simulink model "REFvsFI"  (R2023a)
settings: Solver=FixedStepAuto  StartTime=0.0  StopTime=T  RelTol=1e-3  EnableMultiTasking=on
values from neighbouring files (symbols this model uses):
  Ts = 1    [TestDataGen.m]
libraries: My_FI_Operations x114, simulink x2
(part 2 of 5)

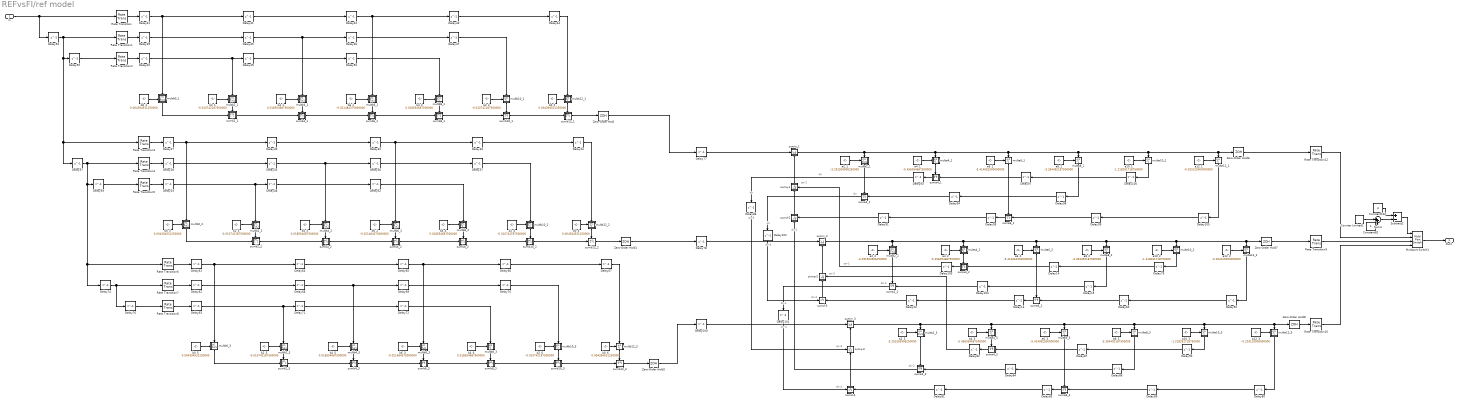
== system REFvsFI/ref model ==
  note: dn-1
  note: dn-2
  note: qn-3
  note: dn-3
  note: qn
  note: dn
  note: dn-4
  note: dn-2
  note: dn-1
  note: qn
  note: dn-4
  note: dn
  note: dn-3
  note: qn-2
  note: qn-3
  note: qn-1
  note: qn-1
  in : Inport
  Constant102 : Constant  Value=4
  Constant82 : Constant
  Counter Limited1 : simulink/Sources/Counter Limited  uplimit=2  tsamp=Ts
  Delay{13..15,23,27..37,39..50,52,60..72,75,77..78,80..82,84..95,97..105,109} (69 alike) : Delay  DelayLength=1  SampleTime=3*Ts
  Delay{53,55,57,59,74,76} (6 alike) : Delay  DelayLength=1  SampleTime=Ts
  Multiport Switch1 : MultiPortSwitch  OutDataTypeStr=double  RndMeth=Nearest  SaturateOnIntegerOverflow=off  InputSameDT=off
  Rate Transition{,1..8} (9 alike) : RateTransition  OutPortSampleTime=3*Ts
  Rate Transition10 : RateTransition  OutPortSampleTime=Ts
  Rate Transition12 : RateTransition  OutPortSampleTime=Ts
  Rate Transition9 : RateTransition  OutPortSampleTime=Ts
  Subtract2 : Sum  Inputs=+-
  Sum4 : Sum  Inputs=|++
  Zero-Order Hold{,1..2,6..8} (6 alike) : ZeroOrderHold  SampleTime=3*Ts
  a10_1 : Constant  Value=-1.218261718750000  OutDataTypeStr=double
  a10_2 : Constant  Value=-1.218261718750000  OutDataTypeStr=double
  a10_3 : Constant  Value=-1.218261718750000  OutDataTypeStr=double
  a12_1 : Constant  Value=-0.203125000000000  OutDataTypeStr=double
  a12_2 : Constant  Value=-0.203125000000000  OutDataTypeStr=double
  a12_3 : Constant  Value=-0.203125000000000  OutDataTypeStr=double
  a2_1 : Constant  Value=-3.291503906250000  OutDataTypeStr=double
  a2_2 : Constant  Value=-3.291503906250000  OutDataTypeStr=double
  a2_3 : Constant  Value=-3.291503906250000  OutDataTypeStr=double
  a4_1 : Constant  Value=-5.456054687500000  OutDataTypeStr=double
  a4_2 : Constant  Value=-5.456054687500000  OutDataTypeStr=double
  a4_3 : Constant  Value=-5.456054687500000  OutDataTypeStr=double
  a6_1 : Constant  Value=-5.414062500000000  OutDataTypeStr=double
  a6_2 : Constant  Value=-5.414062500000000  OutDataTypeStr=double
  a6_3 : Constant  Value=-5.414062500000000  OutDataTypeStr=double
  a8_1 : Constant  Value=-3.354492187500000  OutDataTypeStr=double
  a8_2 : Constant  Value=-3.354492187500000  OutDataTypeStr=double
  a8_3 : Constant  Value=-3.354492187500000  OutDataTypeStr=double
  b0_{1..6} (6 alike) : Constant  Value=0.004394531250000  OutDataTypeStr=double
  b2_{1..6} (6 alike) : Constant  Value=-0.010742187500000  OutDataTypeStr=double
  b4_{1..6} (6 alike) : Constant  Value=0.018554687500000  OutDataTypeStr=double
  b6_1 : Constant  Value=-0.021484375000000  OutDataTypeStr=double
  b6_2 : Constant  Value=-0.021484375000000  OutDataTypeStr=double
  b6_3 : Constant  Value=-0.021484375000000  OutDataTypeStr=double
  multa10_1 : Subsystem  AncestorBlock=My_FI_Operations/multa10_
      settings: LibrarySourceBlock=My_FI_Operations/multa10_  PortSchema="{\"entries\":[{\"content\":{\"sides\":[{\"content\":{\"connectorIds\":[\"In1\"]},\"type\":\"ConnectorPlacement.EquallySpacedRectSide\",\"uuid\":\"423828e0-6700-4575-ac06-a5fb7cb5569f\"},{\"content\":{\"connectorIds\":[],\"side\":\"RIGHT\"},\"type\":\"ConnectorPlacement.EquallySpacedRectSide\",\"uuid\":\"a42db842-eb55-44f2-8f04-0144bc45d908\"},{\"content\":{\"connectorIds\":[\"In2\"],\"side\":\"TOP\"},\"type\":\"ConnectorPlacement.EquallySpacedRectSide\",\"uuid\":\"eef5137d-31f0-46b4-a53b-5aa31464a7f9\"},{\"content\":{\"connectorIds\":[\"Out1\"],\"side\":\"BOTTOM\"},\"type\":\"ConnectorPlacement.EquallySpacedRectSide\",\"uuid\":\"0c804fa9-8d94-49f3-91d8-5fb511150c33\"}]},\"type\":\"ConnectorPlacement.EquallySpacedConnector\",\"uuid\":\"7dd7fe03-b221-4701-a7b2-6552f08320da\"}],\"packageUris\":[\"http://schema.mathworks.com/mf0/Connector/R2020b\"],\"version\":\"1.0\"}"
      mask Display: disp('x')
  multa10_2 : Subsystem  AncestorBlock=My_FI_Operations/multa10_
      settings: LibrarySourceBlock=My_FI_Operations/multa10_  PortSchema="{\"entries\":[{\"content\":{\"sides\":[{\"content\":{\"connectorIds\":[\"In1\"]},\"type\":\"ConnectorPlacement.EquallySpacedRectSide\",\"uuid\":\"423828e0-6700-4575-ac06-a5fb7cb5569f\"},{\"content\":{\"connectorIds\":[],\"side\":\"RIGHT\"},\"type\":\"ConnectorPlacement.EquallySpacedRectSide\",\"uuid\":\"a42db842-eb55-44f2-8f04-0144bc45d908\"},{\"content\":{\"connectorIds\":[\"In2\"],\"side\":\"TOP\"},\"type\":\"ConnectorPlacement.EquallySpacedRectSide\",\"uuid\":\"eef5137d-31f0-46b4-a53b-5aa31464a7f9\"},{\"content\":{\"connectorIds\":[\"Out1\"],\"side\":\"BOTTOM\"},\"type\":\"ConnectorPlacement.EquallySpacedRectSide\",\"uuid\":\"0c804fa9-8d94-49f3-91d8-5fb511150c33\"}]},\"type\":\"ConnectorPlacement.EquallySpacedConnector\",\"uuid\":\"7dd7fe03-b221-4701-a7b2-6552f08320da\"}],\"packageUris\":[\"http://schema.mathworks.com/mf0/Connector/R2020b\"],\"version\":\"1.0\"}"
      mask Display: disp('x')
  multa10_3 : Subsystem  AncestorBlock=My_FI_Operations/multa10_
      settings: LibrarySourceBlock=My_FI_Operations/multa10_  PortSchema="{\"entries\":[{\"content\":{\"sides\":[{\"content\":{\"connectorIds\":[\"In1\"]},\"type\":\"ConnectorPlacement.EquallySpacedRectSide\",\"uuid\":\"423828e0-6700-4575-ac06-a5fb7cb5569f\"},{\"content\":{\"connectorIds\":[],\"side\":\"RIGHT\"},\"type\":\"ConnectorPlacement.EquallySpacedRectSide\",\"uuid\":\"a42db842-eb55-44f2-8f04-0144bc45d908\"},{\"content\":{\"connectorIds\":[\"In2\"],\"side\":\"TOP\"},\"type\":\"ConnectorPlacement.EquallySpacedRectSide\",\"uuid\":\"eef5137d-31f0-46b4-a53b-5aa31464a7f9\"},{\"content\":{\"connectorIds\":[\"Out1\"],\"side\":\"BOTTOM\"},\"type\":\"ConnectorPlacement.EquallySpacedRectSide\",\"uuid\":\"0c804fa9-8d94-49f3-91d8-5fb511150c33\"}]},\"type\":\"ConnectorPlacement.EquallySpacedConnector\",\"uuid\":\"7dd7fe03-b221-4701-a7b2-6552f08320da\"}],\"packageUris\":[\"http://schema.mathworks.com/mf0/Connector/R2020b\"],\"version\":\"1.0\"}"
      mask Display: disp('x')
  multa12_1 : Subsystem  AncestorBlock=My_FI_Operations/multa12_
      settings: LibrarySourceBlock=My_FI_Operations/multa12_  PortSchema="{\"entries\":[{\"content\":{\"sides\":[{\"content\":{\"connectorIds\":[\"In1\"]},\"type\":\"ConnectorPlacement.EquallySpacedRectSide\",\"uuid\":\"423828e0-6700-4575-ac06-a5fb7cb5569f\"},{\"content\":{\"connectorIds\":[],\"side\":\"RIGHT\"},\"type\":\"ConnectorPlacement.EquallySpacedRectSide\",\"uuid\":\"a42db842-eb55-44f2-8f04-0144bc45d908\"},{\"content\":{\"connectorIds\":[\"In2\"],\"side\":\"TOP\"},\"type\":\"ConnectorPlacement.EquallySpacedRectSide\",\"uuid\":\"eef5137d-31f0-46b4-a53b-5aa31464a7f9\"},{\"content\":{\"connectorIds\":[\"Out1\"],\"side\":\"BOTTOM\"},\"type\":\"ConnectorPlacement.EquallySpacedRectSide\",\"uuid\":\"8449918d-02c6-4967-8b4f-9e277713318d\"}]},\"type\":\"ConnectorPlacement.EquallySpacedConnector\",\"uuid\":\"7dd7fe03-b221-4701-a7b2-6552f08320da\"}],\"packageUris\":[\"http://schema.mathworks.com/mf0/Connector/R2020b\"],\"version\":\"1.0\"}"
      mask Display: disp('x')
  multa12_2 : Subsystem  AncestorBlock=My_FI_Operations/multa12_
      settings: LibrarySourceBlock=My_FI_Operations/multa12_  PortSchema="{\"entries\":[{\"content\":{\"sides\":[{\"content\":{\"connectorIds\":[\"In1\"]},\"type\":\"ConnectorPlacement.EquallySpacedRectSide\",\"uuid\":\"423828e0-6700-4575-ac06-a5fb7cb5569f\"},{\"content\":{\"connectorIds\":[],\"side\":\"RIGHT\"},\"type\":\"ConnectorPlacement.EquallySpacedRectSide\",\"uuid\":\"a42db842-eb55-44f2-8f04-0144bc45d908\"},{\"content\":{\"connectorIds\":[\"In2\"],\"side\":\"TOP\"},\"type\":\"ConnectorPlacement.EquallySpacedRectSide\",\"uuid\":\"eef5137d-31f0-46b4-a53b-5aa31464a7f9\"},{\"content\":{\"connectorIds\":[\"Out1\"],\"side\":\"BOTTOM\"},\"type\":\"ConnectorPlacement.EquallySpacedRectSide\",\"uuid\":\"8449918d-02c6-4967-8b4f-9e277713318d\"}]},\"type\":\"ConnectorPlacement.EquallySpacedConnector\",\"uuid\":\"7dd7fe03-b221-4701-a7b2-6552f08320da\"}],\"packageUris\":[\"http://schema.mathworks.com/mf0/Connector/R2020b\"],\"version\":\"1.0\"}"
      mask Display: disp('x')
  multa12_3 : Subsystem  AncestorBlock=My_FI_Operations/multa12_
      settings: LibrarySourceBlock=My_FI_Operations/multa12_  PortSchema="{\"entries\":[{\"content\":{\"sides\":[{\"content\":{\"connectorIds\":[\"In1\"]},\"type\":\"ConnectorPlacement.EquallySpacedRectSide\",\"uuid\":\"423828e0-6700-4575-ac06-a5fb7cb5569f\"},{\"content\":{\"connectorIds\":[],\"side\":\"RIGHT\"},\"type\":\"ConnectorPlacement.EquallySpacedRectSide\",\"uuid\":\"a42db842-eb55-44f2-8f04-0144bc45d908\"},{\"content\":{\"connectorIds\":[\"In2\"],\"side\":\"TOP\"},\"type\":\"ConnectorPlacement.EquallySpacedRectSide\",\"uuid\":\"eef5137d-31f0-46b4-a53b-5aa31464a7f9\"},{\"content\":{\"connectorIds\":[\"Out1\"],\"side\":\"BOTTOM\"},\"type\":\"ConnectorPlacement.EquallySpacedRectSide\",\"uuid\":\"8449918d-02c6-4967-8b4f-9e277713318d\"}]},\"type\":\"ConnectorPlacement.EquallySpacedConnector\",\"uuid\":\"7dd7fe03-b221-4701-a7b2-6552f08320da\"}],\"packageUris\":[\"http://schema.mathworks.com/mf0/Connector/R2020b\"],\"version\":\"1.0\"}"
      mask Display: disp('x')
  multa2_1 : Subsystem  AncestorBlock=My_FI_Operations/multa2_
      settings: LibrarySourceBlock=My_FI_Operations/multa2_  PortSchema="{\"entries\":[{\"content\":{\"sides\":[{\"content\":{\"connectorIds\":[\"In1\"]},\"type\":\"ConnectorPlacement.EquallySpacedRectSide\",\"uuid\":\"423828e0-6700-4575-ac06-a5fb7cb5569f\"},{\"content\":{\"connectorIds\":[],\"side\":\"RIGHT\"},\"type\":\"ConnectorPlacement.EquallySpacedRectSide\",\"uuid\":\"a42db842-eb55-44f2-8f04-0144bc45d908\"},{\"content\":{\"connectorIds\":[\"In2\"],\"side\":\"TOP\"},\"type\":\"ConnectorPlacement.EquallySpacedRectSide\",\"uuid\":\"eef5137d-31f0-46b4-a53b-5aa31464a7f9\"},{\"content\":{\"connectorIds\":[\"Out1\"],\"side\":\"BOTTOM\"},\"type\":\"ConnectorPlacement.EquallySpacedRectSide\",\"uuid\":\"55d96b2a-2b7e-4fdf-a401-8e78f7d2a1aa\"}]},\"type\":\"ConnectorPlacement.EquallySpacedConnector\",\"uuid\":\"7dd7fe03-b221-4701-a7b2-6552f08320da\"}],\"packageUris\":[\"http://schema.mathworks.com/mf0/Connector/R2020b\"],\"version\":\"1.0\"}"
      mask Display: disp('x')
  multa2_2 : Subsystem  AncestorBlock=My_FI_Operations/multa2_
      settings: LibrarySourceBlock=My_FI_Operations/multa2_  PortSchema="{\"entries\":[{\"content\":{\"sides\":[{\"content\":{\"connectorIds\":[\"In1\"]},\"type\":\"ConnectorPlacement.EquallySpacedRectSide\",\"uuid\":\"423828e0-6700-4575-ac06-a5fb7cb5569f\"},{\"content\":{\"connectorIds\":[],\"side\":\"RIGHT\"},\"type\":\"ConnectorPlacement.EquallySpacedRectSide\",\"uuid\":\"a42db842-eb55-44f2-8f04-0144bc45d908\"},{\"content\":{\"connectorIds\":[\"In2\"],\"side\":\"TOP\"},\"type\":\"ConnectorPlacement.EquallySpacedRectSide\",\"uuid\":\"eef5137d-31f0-46b4-a53b-5aa31464a7f9\"},{\"content\":{\"connectorIds\":[\"Out1\"],\"side\":\"BOTTOM\"},\"type\":\"ConnectorPlacement.EquallySpacedRectSide\",\"uuid\":\"55d96b2a-2b7e-4fdf-a401-8e78f7d2a1aa\"}]},\"type\":\"ConnectorPlacement.EquallySpacedConnector\",\"uuid\":\"7dd7fe03-b221-4701-a7b2-6552f08320da\"}],\"packageUris\":[\"http://schema.mathworks.com/mf0/Connector/R2020b\"],\"version\":\"1.0\"}"
      mask Display: disp('x')
  multa2_3 : Subsystem  AncestorBlock=My_FI_Operations/multa2_
      settings: LibrarySourceBlock=My_FI_Operations/multa2_  PortSchema="{\"entries\":[{\"content\":{\"sides\":[{\"content\":{\"connectorIds\":[\"In1\"]},\"type\":\"ConnectorPlacement.EquallySpacedRectSide\",\"uuid\":\"423828e0-6700-4575-ac06-a5fb7cb5569f\"},{\"content\":{\"connectorIds\":[],\"side\":\"RIGHT\"},\"type\":\"ConnectorPlacement.EquallySpacedRectSide\",\"uuid\":\"a42db842-eb55-44f2-8f04-0144bc45d908\"},{\"content\":{\"connectorIds\":[\"In2\"],\"side\":\"TOP\"},\"type\":\"ConnectorPlacement.EquallySpacedRectSide\",\"uuid\":\"eef5137d-31f0-46b4-a53b-5aa31464a7f9\"},{\"content\":{\"connectorIds\":[\"Out1\"],\"side\":\"BOTTOM\"},\"type\":\"ConnectorPlacement.EquallySpacedRectSide\",\"uuid\":\"55d96b2a-2b7e-4fdf-a401-8e78f7d2a1aa\"}]},\"type\":\"ConnectorPlacement.EquallySpacedConnector\",\"uuid\":\"7dd7fe03-b221-4701-a7b2-6552f08320da\"}],\"packageUris\":[\"http://schema.mathworks.com/mf0/Connector/R2020b\"],\"version\":\"1.0\"}"
      mask Display: disp('x')
  multa4_1 : Subsystem  AncestorBlock=My_FI_Operations/multa4_
      settings: LibrarySourceBlock=My_FI_Operations/multa4_  PortSchema="{\"entries\":[{\"content\":{\"sides\":[{\"content\":{\"connectorIds\":[\"In1\"]},\"type\":\"ConnectorPlacement.EquallySpacedRectSide\",\"uuid\":\"423828e0-6700-4575-ac06-a5fb7cb5569f\"},{\"content\":{\"connectorIds\":[],\"side\":\"RIGHT\"},\"type\":\"ConnectorPlacement.EquallySpacedRectSide\",\"uuid\":\"a42db842-eb55-44f2-8f04-0144bc45d908\"},{\"content\":{\"connectorIds\":[\"In2\"],\"side\":\"TOP\"},\"type\":\"ConnectorPlacement.EquallySpacedRectSide\",\"uuid\":\"eef5137d-31f0-46b4-a53b-5aa31464a7f9\"},{\"content\":{\"connectorIds\":[\"Out1\"],\"side\":\"BOTTOM\"},\"type\":\"ConnectorPlacement.EquallySpacedRectSide\",\"uuid\":\"24a9476e-4370-431a-bbc5-245c90c7a6e7\"}]},\"type\":\"ConnectorPlacement.EquallySpacedConnector\",\"uuid\":\"7dd7fe03-b221-4701-a7b2-6552f08320da\"}],\"packageUris\":[\"http://schema.mathworks.com/mf0/Connector/R2020b\"],\"version\":\"1.0\"}"
      mask Display: disp('x')
  multa4_2 : Subsystem  AncestorBlock=My_FI_Operations/multa4_
      settings: LibrarySourceBlock=My_FI_Operations/multa4_  PortSchema="{\"entries\":[{\"content\":{\"sides\":[{\"content\":{\"connectorIds\":[\"In1\"]},\"type\":\"ConnectorPlacement.EquallySpacedRectSide\",\"uuid\":\"423828e0-6700-4575-ac06-a5fb7cb5569f\"},{\"content\":{\"connectorIds\":[],\"side\":\"RIGHT\"},\"type\":\"ConnectorPlacement.EquallySpacedRectSide\",\"uuid\":\"a42db842-eb55-44f2-8f04-0144bc45d908\"},{\"content\":{\"connectorIds\":[\"In2\"],\"side\":\"TOP\"},\"type\":\"ConnectorPlacement.EquallySpacedRectSide\",\"uuid\":\"eef5137d-31f0-46b4-a53b-5aa31464a7f9\"},{\"content\":{\"connectorIds\":[\"Out1\"],\"side\":\"BOTTOM\"},\"type\":\"ConnectorPlacement.EquallySpacedRectSide\",\"uuid\":\"24a9476e-4370-431a-bbc5-245c90c7a6e7\"}]},\"type\":\"ConnectorPlacement.EquallySpacedConnector\",\"uuid\":\"7dd7fe03-b221-4701-a7b2-6552f08320da\"}],\"packageUris\":[\"http://schema.mathworks.com/mf0/Connector/R2020b\"],\"version\":\"1.0\"}"
      mask Display: disp('x')
  multa4_3 : Subsystem  AncestorBlock=My_FI_Operations/multa4_
      settings: LibrarySourceBlock=My_FI_Operations/multa4_  PortSchema="{\"entries\":[{\"content\":{\"sides\":[{\"content\":{\"connectorIds\":[\"In1\"]},\"type\":\"ConnectorPlacement.EquallySpacedRectSide\",\"uuid\":\"423828e0-6700-4575-ac06-a5fb7cb5569f\"},{\"content\":{\"connectorIds\":[],\"side\":\"RIGHT\"},\"type\":\"ConnectorPlacement.EquallySpacedRectSide\",\"uuid\":\"a42db842-eb55-44f2-8f04-0144bc45d908\"},{\"content\":{\"connectorIds\":[\"In2\"],\"side\":\"TOP\"},\"type\":\"ConnectorPlacement.EquallySpacedRectSide\",\"uuid\":\"eef5137d-31f0-46b4-a53b-5aa31464a7f9\"},{\"content\":{\"connectorIds\":[\"Out1\"],\"side\":\"BOTTOM\"},\"type\":\"ConnectorPlacement.EquallySpacedRectSide\",\"uuid\":\"24a9476e-4370-431a-bbc5-245c90c7a6e7\"}]},\"type\":\"ConnectorPlacement.EquallySpacedConnector\",\"uuid\":\"7dd7fe03-b221-4701-a7b2-6552f08320da\"}],\"packageUris\":[\"http://schema.mathworks.com/mf0/Connector/R2020b\"],\"version\":\"1.0\"}"
      mask Display: disp('x')
  multa6_1 : Subsystem  AncestorBlock=My_FI_Operations/multa6_
      settings: LibrarySourceBlock=My_FI_Operations/multa6_  PortSchema="{\"entries\":[{\"content\":{\"sides\":[{\"content\":{\"connectorIds\":[\"In1\"]},\"type\":\"ConnectorPlacement.EquallySpacedRectSide\",\"uuid\":\"423828e0-6700-4575-ac06-a5fb7cb5569f\"},{\"content\":{\"connectorIds\":[],\"side\":\"RIGHT\"},\"type\":\"ConnectorPlacement.EquallySpacedRectSide\",\"uuid\":\"a42db842-eb55-44f2-8f04-0144bc45d908\"},{\"content\":{\"connectorIds\":[\"In2\"],\"side\":\"TOP\"},\"type\":\"ConnectorPlacement.EquallySpacedRectSide\",\"uuid\":\"eef5137d-31f0-46b4-a53b-5aa31464a7f9\"},{\"content\":{\"connectorIds\":[\"Out1\"],\"side\":\"BOTTOM\"},\"type\":\"ConnectorPlacement.EquallySpacedRectSide\",\"uuid\":\"47329aef-84bb-47a0-9b32-b12909a392a1\"}]},\"type\":\"ConnectorPlacement.EquallySpacedConnector\",\"uuid\":\"7dd7fe03-b221-4701-a7b2-6552f08320da\"}],\"packageUris\":[\"http://schema.mathworks.com/mf0/Connector/R2020b\"],\"version\":\"1.0\"}"
      mask Display: disp('x')
  multa6_2 : Subsystem  AncestorBlock=My_FI_Operations/multa6_
      settings: LibrarySourceBlock=My_FI_Operations/multa6_  PortSchema="{\"entries\":[{\"content\":{\"sides\":[{\"content\":{\"connectorIds\":[\"In1\"]},\"type\":\"ConnectorPlacement.EquallySpacedRectSide\",\"uuid\":\"423828e0-6700-4575-ac06-a5fb7cb5569f\"},{\"content\":{\"connectorIds\":[],\"side\":\"RIGHT\"},\"type\":\"ConnectorPlacement.EquallySpacedRectSide\",\"uuid\":\"a42db842-eb55-44f2-8f04-0144bc45d908\"},{\"content\":{\"connectorIds\":[\"In2\"],\"side\":\"TOP\"},\"type\":\"ConnectorPlacement.EquallySpacedRectSide\",\"uuid\":\"eef5137d-31f0-46b4-a53b-5aa31464a7f9\"},{\"content\":{\"connectorIds\":[\"Out1\"],\"side\":\"BOTTOM\"},\"type\":\"ConnectorPlacement.EquallySpacedRectSide\",\"uuid\":\"47329aef-84bb-47a0-9b32-b12909a392a1\"}]},\"type\":\"ConnectorPlacement.EquallySpacedConnector\",\"uuid\":\"7dd7fe03-b221-4701-a7b2-6552f08320da\"}],\"packageUris\":[\"http://schema.mathworks.com/mf0/Connector/R2020b\"],\"version\":\"1.0\"}"
      mask Display: disp('x')
  multa6_3 : Subsystem  AncestorBlock=My_FI_Operations/multa6_
      settings: LibrarySourceBlock=My_FI_Operations/multa6_  PortSchema="{\"entries\":[{\"content\":{\"sides\":[{\"content\":{\"connectorIds\":[\"In1\"]},\"type\":\"ConnectorPlacement.EquallySpacedRectSide\",\"uuid\":\"423828e0-6700-4575-ac06-a5fb7cb5569f\"},{\"content\":{\"connectorIds\":[],\"side\":\"RIGHT\"},\"type\":\"ConnectorPlacement.EquallySpacedRectSide\",\"uuid\":\"a42db842-eb55-44f2-8f04-0144bc45d908\"},{\"content\":{\"connectorIds\":[\"In2\"],\"side\":\"TOP\"},\"type\":\"ConnectorPlacement.EquallySpacedRectSide\",\"uuid\":\"eef5137d-31f0-46b4-a53b-5aa31464a7f9\"},{\"content\":{\"connectorIds\":[\"Out1\"],\"side\":\"BOTTOM\"},\"type\":\"ConnectorPlacement.EquallySpacedRectSide\",\"uuid\":\"47329aef-84bb-47a0-9b32-b12909a392a1\"}]},\"type\":\"ConnectorPlacement.EquallySpacedConnector\",\"uuid\":\"7dd7fe03-b221-4701-a7b2-6552f08320da\"}],\"packageUris\":[\"http://schema.mathworks.com/mf0/Connector/R2020b\"],\"version\":\"1.0\"}"
      mask Display: disp('x')
  multa8_1 : Subsystem  AncestorBlock=My_FI_Operations/multa8_
      settings: LibrarySourceBlock=My_FI_Operations/multa8_  PortSchema="{\"entries\":[{\"content\":{\"sides\":[{\"content\":{\"connectorIds\":[\"In1\"]},\"type\":\"ConnectorPlacement.EquallySpacedRectSide\",\"uuid\":\"423828e0-6700-4575-ac06-a5fb7cb5569f\"},{\"content\":{\"connectorIds\":[],\"side\":\"RIGHT\"},\"type\":\"ConnectorPlacement.EquallySpacedRectSide\",\"uuid\":\"a42db842-eb55-44f2-8f04-0144bc45d908\"},{\"content\":{\"connectorIds\":[\"In2\"],\"side\":\"TOP\"},\"type\":\"ConnectorPlacement.EquallySpacedRectSide\",\"uuid\":\"eef5137d-31f0-46b4-a53b-5aa31464a7f9\"},{\"content\":{\"connectorIds\":[\"Out1\"],\"side\":\"BOTTOM\"},\"type\":\"ConnectorPlacement.EquallySpacedRectSide\",\"uuid\":\"5c073f60-f22f-4cd7-abc5-d0d5f88f0213\"}]},\"type\":\"ConnectorPlacement.EquallySpacedConnector\",\"uuid\":\"7dd7fe03-b221-4701-a7b2-6552f08320da\"}],\"packageUris\":[\"http://schema.mathworks.com/mf0/Connector/R2020b\"],\"version\":\"1.0\"}"
      mask Display: disp('x')
  multa8_2 : Subsystem  AncestorBlock=My_FI_Operations/multa8_
      settings: LibrarySourceBlock=My_FI_Operations/multa8_  PortSchema="{\"entries\":[{\"content\":{\"sides\":[{\"content\":{\"connectorIds\":[\"In1\"]},\"type\":\"ConnectorPlacement.EquallySpacedRectSide\",\"uuid\":\"423828e0-6700-4575-ac06-a5fb7cb5569f\"},{\"content\":{\"connectorIds\":[],\"side\":\"RIGHT\"},\"type\":\"ConnectorPlacement.EquallySpacedRectSide\",\"uuid\":\"a42db842-eb55-44f2-8f04-0144bc45d908\"},{\"content\":{\"connectorIds\":[\"In2\"],\"side\":\"TOP\"},\"type\":\"ConnectorPlacement.EquallySpacedRectSide\",\"uuid\":\"eef5137d-31f0-46b4-a53b-5aa31464a7f9\"},{\"content\":{\"connectorIds\":[\"Out1\"],\"side\":\"BOTTOM\"},\"type\":\"ConnectorPlacement.EquallySpacedRectSide\",\"uuid\":\"5c073f60-f22f-4cd7-abc5-d0d5f88f0213\"}]},\"type\":\"ConnectorPlacement.EquallySpacedConnector\",\"uuid\":\"7dd7fe03-b221-4701-a7b2-6552f08320da\"}],\"packageUris\":[\"http://schema.mathworks.com/mf0/Connector/R2020b\"],\"version\":\"1.0\"}"
      mask Display: disp('x')
  multa8_3 : Subsystem  AncestorBlock=My_FI_Operations/multa8_
      settings: LibrarySourceBlock=My_FI_Operations/multa8_  PortSchema="{\"entries\":[{\"content\":{\"sides\":[{\"content\":{\"connectorIds\":[\"In1\"]},\"type\":\"ConnectorPlacement.EquallySpacedRectSide\",\"uuid\":\"423828e0-6700-4575-ac06-a5fb7cb5569f\"},{\"content\":{\"connectorIds\":[],\"side\":\"RIGHT\"},\"type\":\"ConnectorPlacement.EquallySpacedRectSide\",\"uuid\":\"a42db842-eb55-44f2-8f04-0144bc45d908\"},{\"content\":{\"connectorIds\":[\"In2\"],\"side\":\"TOP\"},\"type\":\"ConnectorPlacement.EquallySpacedRectSide\",\"uuid\":\"eef5137d-31f0-46b4-a53b-5aa31464a7f9\"},{\"content\":{\"connectorIds\":[\"Out1\"],\"side\":\"BOTTOM\"},\"type\":\"ConnectorPlacement.EquallySpacedRectSide\",\"uuid\":\"5c073f60-f22f-4cd7-abc5-d0d5f88f0213\"}]},\"type\":\"ConnectorPlacement.EquallySpacedConnector\",\"uuid\":\"7dd7fe03-b221-4701-a7b2-6552f08320da\"}],\"packageUris\":[\"http://schema.mathworks.com/mf0/Connector/R2020b\"],\"version\":\"1.0\"}"
      mask Display: disp('x')
  multb0_1 : Subsystem  AncestorBlock=My_FI_Operations/multb0_
      settings: LibrarySourceBlock=My_FI_Operations/multb0_  PortSchema="{\"entries\":[{\"content\":{\"sides\":[{\"content\":{\"connectorIds\":[\"In1\"]},\"type\":\"ConnectorPlacement.EquallySpacedRectSide\",\"uuid\":\"20461ecc-945a-453b-bec8-f18bcbd4d7ca\"},{\"content\":{\"connectorIds\":[],\"side\":\"RIGHT\"},\"type\":\"ConnectorPlacement.EquallySpacedRectSide\",\"uuid\":\"a806ae65-26a1-4387-823f-a90265b6c751\"},{\"content\":{\"connectorIds\":[\"In2\"],\"side\":\"TOP\"},\"type\":\"ConnectorPlacement.EquallySpacedRectSide\",\"uuid\":\"faa34e1a-fdc6-4b39-b604-acf00955d353\"},{\"content\":{\"connectorIds\":[\"Out1\"],\"side\":\"BOTTOM\"},\"type\":\"ConnectorPlacement.EquallySpacedRectSide\",\"uuid\":\"6d48c7d1-ec45-4610-bf5d-3af7cf103011\"}]},\"type\":\"ConnectorPlacement.EquallySpacedConnector\",\"uuid\":\"f3c21808-e34e-4785-8275-0070ba5b450f\"}],\"packageUris\":[\"http://schema.mathworks.com/mf0/Connector/R2020b\"],\"version\":\"1.0\"}"
      mask Display: disp('x')
  multb0_2 : Subsystem  AncestorBlock=My_FI_Operations/multb0_
      settings: LibrarySourceBlock=My_FI_Operations/multb0_  PortSchema="{\"entries\":[{\"content\":{\"sides\":[{\"content\":{\"connectorIds\":[\"In1\"]},\"type\":\"ConnectorPlacement.EquallySpacedRectSide\",\"uuid\":\"20461ecc-945a-453b-bec8-f18bcbd4d7ca\"},{\"content\":{\"connectorIds\":[],\"side\":\"RIGHT\"},\"type\":\"ConnectorPlacement.EquallySpacedRectSide\",\"uuid\":\"a806ae65-26a1-4387-823f-a90265b6c751\"},{\"content\":{\"connectorIds\":[\"In2\"],\"side\":\"TOP\"},\"type\":\"ConnectorPlacement.EquallySpacedRectSide\",\"uuid\":\"faa34e1a-fdc6-4b39-b604-acf00955d353\"},{\"content\":{\"connectorIds\":[\"Out1\"],\"side\":\"BOTTOM\"},\"type\":\"ConnectorPlacement.EquallySpacedRectSide\",\"uuid\":\"6d48c7d1-ec45-4610-bf5d-3af7cf103011\"}]},\"type\":\"ConnectorPlacement.EquallySpacedConnector\",\"uuid\":\"f3c21808-e34e-4785-8275-0070ba5b450f\"}],\"packageUris\":[\"http://schema.mathworks.com/mf0/Connector/R2020b\"],\"version\":\"1.0\"}"
      mask Display: disp('x')
  multb0_3 : Subsystem  AncestorBlock=My_FI_Operations/multb0_
      settings: LibrarySourceBlock=My_FI_Operations/multb0_  PortSchema="{\"entries\":[{\"content\":{\"sides\":[{\"content\":{\"connectorIds\":[\"In1\"]},\"type\":\"ConnectorPlacement.EquallySpacedRectSide\",\"uuid\":\"20461ecc-945a-453b-bec8-f18bcbd4d7ca\"},{\"content\":{\"connectorIds\":[],\"side\":\"RIGHT\"},\"type\":\"ConnectorPlacement.EquallySpacedRectSide\",\"uuid\":\"a806ae65-26a1-4387-823f-a90265b6c751\"},{\"content\":{\"connectorIds\":[\"In2\"],\"side\":\"TOP\"},\"type\":\"ConnectorPlacement.EquallySpacedRectSide\",\"uuid\":\"faa34e1a-fdc6-4b39-b604-acf00955d353\"},{\"content\":{\"connectorIds\":[\"Out1\"],\"side\":\"BOTTOM\"},\"type\":\"ConnectorPlacement.EquallySpacedRectSide\",\"uuid\":\"6d48c7d1-ec45-4610-bf5d-3af7cf103011\"}]},\"type\":\"ConnectorPlacement.EquallySpacedConnector\",\"uuid\":\"f3c21808-e34e-4785-8275-0070ba5b450f\"}],\"packageUris\":[\"http://schema.mathworks.com/mf0/Connector/R2020b\"],\"version\":\"1.0\"}"
      mask Display: disp('x')
  multb10_1 : Subsystem  AncestorBlock=My_FI_Operations/multb10_
      settings: LibrarySourceBlock=My_FI_Operations/multb10_  PortSchema="{\"entries\":[{\"content\":{\"sides\":[{\"content\":{\"connectorIds\":[\"In1\"]},\"type\":\"ConnectorPlacement.EquallySpacedRectSide\",\"uuid\":\"20461ecc-945a-453b-bec8-f18bcbd4d7ca\"},{\"content\":{\"connectorIds\":[],\"side\":\"RIGHT\"},\"type\":\"ConnectorPlacement.EquallySpacedRectSide\",\"uuid\":\"a806ae65-26a1-4387-823f-a90265b6c751\"},{\"content\":{\"connectorIds\":[\"In2\"],\"side\":\"TOP\"},\"type\":\"ConnectorPlacement.EquallySpacedRectSide\",\"uuid\":\"faa34e1a-fdc6-4b39-b604-acf00955d353\"},{\"content\":{\"connectorIds\":[\"Out1\"],\"side\":\"BOTTOM\"},\"type\":\"ConnectorPlacement.EquallySpacedRectSide\",\"uuid\":\"227775b0-b587-499e-95de-63528f3ed159\"}]},\"type\":\"ConnectorPlacement.EquallySpacedConnector\",\"uuid\":\"f3c21808-e34e-4785-8275-0070ba5b450f\"}],\"packageUris\":[\"http://schema.mathworks.com/mf0/Connector/R2020b\"],\"version\":\"1.0\"}"
      mask Display: disp('x')
  multb10_2 : Subsystem  AncestorBlock=My_FI_Operations/multb10_
      settings: LibrarySourceBlock=My_FI_Operations/multb10_  PortSchema="{\"entries\":[{\"content\":{\"sides\":[{\"content\":{\"connectorIds\":[\"In1\"]},\"type\":\"ConnectorPlacement.EquallySpacedRectSide\",\"uuid\":\"20461ecc-945a-453b-bec8-f18bcbd4d7ca\"},{\"content\":{\"connectorIds\":[],\"side\":\"RIGHT\"},\"type\":\"ConnectorPlacement.EquallySpacedRectSide\",\"uuid\":\"a806ae65-26a1-4387-823f-a90265b6c751\"},{\"content\":{\"connectorIds\":[\"In2\"],\"side\":\"TOP\"},\"type\":\"ConnectorPlacement.EquallySpacedRectSide\",\"uuid\":\"faa34e1a-fdc6-4b39-b604-acf00955d353\"},{\"content\":{\"connectorIds\":[\"Out1\"],\"side\":\"BOTTOM\"},\"type\":\"ConnectorPlacement.EquallySpacedRectSide\",\"uuid\":\"227775b0-b587-499e-95de-63528f3ed159\"}]},\"type\":\"ConnectorPlacement.EquallySpacedConnector\",\"uuid\":\"f3c21808-e34e-4785-8275-0070ba5b450f\"}],\"packageUris\":[\"http://schema.mathworks.com/mf0/Connector/R2020b\"],\"version\":\"1.0\"}"
      mask Display: disp('x')
  multb10_3 : Subsystem  AncestorBlock=My_FI_Operations/multb10_
      settings: LibrarySourceBlock=My_FI_Operations/multb10_  PortSchema="{\"entries\":[{\"content\":{\"sides\":[{\"content\":{\"connectorIds\":[\"In1\"]},\"type\":\"ConnectorPlacement.EquallySpacedRectSide\",\"uuid\":\"20461ecc-945a-453b-bec8-f18bcbd4d7ca\"},{\"content\":{\"connectorIds\":[],\"side\":\"RIGHT\"},\"type\":\"ConnectorPlacement.EquallySpacedRectSide\",\"uuid\":\"a806ae65-26a1-4387-823f-a90265b6c751\"},{\"content\":{\"connectorIds\":[\"In2\"],\"side\":\"TOP\"},\"type\":\"ConnectorPlacement.EquallySpacedRectSide\",\"uuid\":\"faa34e1a-fdc6-4b39-b604-acf00955d353\"},{\"content\":{\"connectorIds\":[\"Out1\"],\"side\":\"BOTTOM\"},\"type\":\"ConnectorPlacement.EquallySpacedRectSide\",\"uuid\":\"227775b0-b587-499e-95de-63528f3ed159\"}]},\"type\":\"ConnectorPlacement.EquallySpacedConnector\",\"uuid\":\"f3c21808-e34e-4785-8275-0070ba5b450f\"}],\"packageUris\":[\"http://schema.mathworks.com/mf0/Connector/R2020b\"],\"version\":\"1.0\"}"
      mask Display: disp('x')
  multb12_1 : Subsystem  AncestorBlock=My_FI_Operations/multb12_
      settings: LibrarySourceBlock=My_FI_Operations/multb12_  PortSchema="{\"entries\":[{\"content\":{\"sides\":[{\"content\":{\"connectorIds\":[\"In1\"]},\"type\":\"ConnectorPlacement.EquallySpacedRectSide\",\"uuid\":\"20461ecc-945a-453b-bec8-f18bcbd4d7ca\"},{\"content\":{\"connectorIds\":[],\"side\":\"RIGHT\"},\"type\":\"ConnectorPlacement.EquallySpacedRectSide\",\"uuid\":\"a806ae65-26a1-4387-823f-a90265b6c751\"},{\"content\":{\"connectorIds\":[\"In2\"],\"side\":\"TOP\"},\"type\":\"ConnectorPlacement.EquallySpacedRectSide\",\"uuid\":\"faa34e1a-fdc6-4b39-b604-acf00955d353\"},{\"content\":{\"connectorIds\":[\"Out1\"],\"side\":\"BOTTOM\"},\"type\":\"ConnectorPlacement.EquallySpacedRectSide\",\"uuid\":\"38ae6b7a-ab73-4307-ae98-7ba73f698229\"}]},\"type\":\"ConnectorPlacement.EquallySpacedConnector\",\"uuid\":\"f3c21808-e34e-4785-8275-0070ba5b450f\"}],\"packageUris\":[\"http://schema.mathworks.com/mf0/Connector/R2020b\"],\"version\":\"1.0\"}"
      mask Display: disp('x')
  multb12_2 : Subsystem  AncestorBlock=My_FI_Operations/multb12_
      settings: LibrarySourceBlock=My_FI_Operations/multb12_  PortSchema="{\"entries\":[{\"content\":{\"sides\":[{\"content\":{\"connectorIds\":[\"In1\"]},\"type\":\"ConnectorPlacement.EquallySpacedRectSide\",\"uuid\":\"20461ecc-945a-453b-bec8-f18bcbd4d7ca\"},{\"content\":{\"connectorIds\":[],\"side\":\"RIGHT\"},\"type\":\"ConnectorPlacement.EquallySpacedRectSide\",\"uuid\":\"a806ae65-26a1-4387-823f-a90265b6c751\"},{\"content\":{\"connectorIds\":[\"In2\"],\"side\":\"TOP\"},\"type\":\"ConnectorPlacement.EquallySpacedRectSide\",\"uuid\":\"faa34e1a-fdc6-4b39-b604-acf00955d353\"},{\"content\":{\"connectorIds\":[\"Out1\"],\"side\":\"BOTTOM\"},\"type\":\"ConnectorPlacement.EquallySpacedRectSide\",\"uuid\":\"38ae6b7a-ab73-4307-ae98-7ba73f698229\"}]},\"type\":\"ConnectorPlacement.EquallySpacedConnector\",\"uuid\":\"f3c21808-e34e-4785-8275-0070ba5b450f\"}],\"packageUris\":[\"http://schema.mathworks.com/mf0/Connector/R2020b\"],\"version\":\"1.0\"}"
      mask Display: disp('x')
  multb12_3 : Subsystem  AncestorBlock=My_FI_Operations/multb12_
      settings: LibrarySourceBlock=My_FI_Operations/multb12_  PortSchema="{\"entries\":[{\"content\":{\"sides\":[{\"content\":{\"connectorIds\":[\"In1\"]},\"type\":\"ConnectorPlacement.EquallySpacedRectSide\",\"uuid\":\"20461ecc-945a-453b-bec8-f18bcbd4d7ca\"},{\"content\":{\"connectorIds\":[],\"side\":\"RIGHT\"},\"type\":\"ConnectorPlacement.EquallySpacedRectSide\",\"uuid\":\"a806ae65-26a1-4387-823f-a90265b6c751\"},{\"content\":{\"connectorIds\":[\"In2\"],\"side\":\"TOP\"},\"type\":\"ConnectorPlacement.EquallySpacedRectSide\",\"uuid\":\"faa34e1a-fdc6-4b39-b604-acf00955d353\"},{\"content\":{\"connectorIds\":[\"Out1\"],\"side\":\"BOTTOM\"},\"type\":\"ConnectorPlacement.EquallySpacedRectSide\",\"uuid\":\"38ae6b7a-ab73-4307-ae98-7ba73f698229\"}]},\"type\":\"ConnectorPlacement.EquallySpacedConnector\",\"uuid\":\"f3c21808-e34e-4785-8275-0070ba5b450f\"}],\"packageUris\":[\"http://schema.mathworks.com/mf0/Connector/R2020b\"],\"version\":\"1.0\"}"
      mask Display: disp('x')
  multb2_1 : Subsystem  AncestorBlock=My_FI_Operations/multb2_
      settings: LibrarySourceBlock=My_FI_Operations/multb2_  PortSchema="{\"entries\":[{\"content\":{\"sides\":[{\"content\":{\"connectorIds\":[\"In1\"]},\"type\":\"ConnectorPlacement.EquallySpacedRectSide\",\"uuid\":\"20461ecc-945a-453b-bec8-f18bcbd4d7ca\"},{\"content\":{\"connectorIds\":[],\"side\":\"RIGHT\"},\"type\":\"ConnectorPlacement.EquallySpacedRectSide\",\"uuid\":\"a806ae65-26a1-4387-823f-a90265b6c751\"},{\"content\":{\"connectorIds\":[\"In2\"],\"side\":\"TOP\"},\"type\":\"ConnectorPlacement.EquallySpacedRectSide\",\"uuid\":\"faa34e1a-fdc6-4b39-b604-acf00955d353\"},{\"content\":{\"connectorIds\":[\"Out1\"],\"side\":\"BOTTOM\"},\"type\":\"ConnectorPlacement.EquallySpacedRectSide\",\"uuid\":\"e1b0fef8-c153-494e-8ffe-3515e962a3c5\"}]},\"type\":\"ConnectorPlacement.EquallySpacedConnector\",\"uuid\":\"f3c21808-e34e-4785-8275-0070ba5b450f\"}],\"packageUris\":[\"http://schema.mathworks.com/mf0/Connector/R2020b\"],\"version\":\"1.0\"}"
      mask Display: disp('x')
  multb2_2 : Subsystem  AncestorBlock=My_FI_Operations/multb2_
      settings: LibrarySourceBlock=My_FI_Operations/multb2_  PortSchema="{\"entries\":[{\"content\":{\"sides\":[{\"content\":{\"connectorIds\":[\"In1\"]},\"type\":\"ConnectorPlacement.EquallySpacedRectSide\",\"uuid\":\"20461ecc-945a-453b-bec8-f18bcbd4d7ca\"},{\"content\":{\"connectorIds\":[],\"side\":\"RIGHT\"},\"type\":\"ConnectorPlacement.EquallySpacedRectSide\",\"uuid\":\"a806ae65-26a1-4387-823f-a90265b6c751\"},{\"content\":{\"connectorIds\":[\"In2\"],\"side\":\"TOP\"},\"type\":\"ConnectorPlacement.EquallySpacedRectSide\",\"uuid\":\"faa34e1a-fdc6-4b39-b604-acf00955d353\"},{\"content\":{\"connectorIds\":[\"Out1\"],\"side\":\"BOTTOM\"},\"type\":\"ConnectorPlacement.EquallySpacedRectSide\",\"uuid\":\"e1b0fef8-c153-494e-8ffe-3515e962a3c5\"}]},\"type\":\"ConnectorPlacement.EquallySpacedConnector\",\"uuid\":\"f3c21808-e34e-4785-8275-0070ba5b450f\"}],\"packageUris\":[\"http://schema.mathworks.com/mf0/Connector/R2020b\"],\"version\":\"1.0\"}"
      mask Display: disp('x')
  multb2_3 : Subsystem  AncestorBlock=My_FI_Operations/multb2_
      settings: LibrarySourceBlock=My_FI_Operations/multb2_  PortSchema="{\"entries\":[{\"content\":{\"sides\":[{\"content\":{\"connectorIds\":[\"In1\"]},\"type\":\"ConnectorPlacement.EquallySpacedRectSide\",\"uuid\":\"20461ecc-945a-453b-bec8-f18bcbd4d7ca\"},{\"content\":{\"connectorIds\":[],\"side\":\"RIGHT\"},\"type\":\"ConnectorPlacement.EquallySpacedRectSide\",\"uuid\":\"a806ae65-26a1-4387-823f-a90265b6c751\"},{\"content\":{\"connectorIds\":[\"In2\"],\"side\":\"TOP\"},\"type\":\"ConnectorPlacement.EquallySpacedRectSide\",\"uuid\":\"faa34e1a-fdc6-4b39-b604-acf00955d353\"},{\"content\":{\"connectorIds\":[\"Out1\"],\"side\":\"BOTTOM\"},\"type\":\"ConnectorPlacement.EquallySpacedRectSide\",\"uuid\":\"e1b0fef8-c153-494e-8ffe-3515e962a3c5\"}]},\"type\":\"ConnectorPlacement.EquallySpacedConnector\",\"uuid\":\"f3c21808-e34e-4785-8275-0070ba5b450f\"}],\"packageUris\":[\"http://schema.mathworks.com/mf0/Connector/R2020b\"],\"version\":\"1.0\"}"
      mask Display: disp('x')
  multb4_1 : Subsystem  AncestorBlock=My_FI_Operations/multb4_
      settings: LibrarySourceBlock=My_FI_Operations/multb4_  PortSchema="{\"entries\":[{\"content\":{\"sides\":[{\"content\":{\"connectorIds\":[\"In1\"]},\"type\":\"ConnectorPlacement.EquallySpacedRectSide\",\"uuid\":\"20461ecc-945a-453b-bec8-f18bcbd4d7ca\"},{\"content\":{\"connectorIds\":[],\"side\":\"RIGHT\"},\"type\":\"ConnectorPlacement.EquallySpacedRectSide\",\"uuid\":\"a806ae65-26a1-4387-823f-a90265b6c751\"},{\"content\":{\"connectorIds\":[\"In2\"],\"side\":\"TOP\"},\"type\":\"ConnectorPlacement.EquallySpacedRectSide\",\"uuid\":\"faa34e1a-fdc6-4b39-b604-acf00955d353\"},{\"content\":{\"connectorIds\":[\"Out1\"],\"side\":\"BOTTOM\"},\"type\":\"ConnectorPlacement.EquallySpacedRectSide\",\"uuid\":\"234e609c-6b95-41af-91dd-8a06091f2e10\"}]},\"type\":\"ConnectorPlacement.EquallySpacedConnector\",\"uuid\":\"f3c21808-e34e-4785-8275-0070ba5b450f\"}],\"packageUris\":[\"http://schema.mathworks.com/mf0/Connector/R2020b\"],\"version\":\"1.0\"}"
      mask Display: disp('x')
  multb4_2 : Subsystem  AncestorBlock=My_FI_Operations/multb4_
      settings: LibrarySourceBlock=My_FI_Operations/multb4_  PortSchema="{\"entries\":[{\"content\":{\"sides\":[{\"content\":{\"connectorIds\":[\"In1\"]},\"type\":\"ConnectorPlacement.EquallySpacedRectSide\",\"uuid\":\"20461ecc-945a-453b-bec8-f18bcbd4d7ca\"},{\"content\":{\"connectorIds\":[],\"side\":\"RIGHT\"},\"type\":\"ConnectorPlacement.EquallySpacedRectSide\",\"uuid\":\"a806ae65-26a1-4387-823f-a90265b6c751\"},{\"content\":{\"connectorIds\":[\"In2\"],\"side\":\"TOP\"},\"type\":\"ConnectorPlacement.EquallySpacedRectSide\",\"uuid\":\"faa34e1a-fdc6-4b39-b604-acf00955d353\"},{\"content\":{\"connectorIds\":[\"Out1\"],\"side\":\"BOTTOM\"},\"type\":\"ConnectorPlacement.EquallySpacedRectSide\",\"uuid\":\"234e609c-6b95-41af-91dd-8a06091f2e10\"}]},\"type\":\"ConnectorPlacement.EquallySpacedConnector\",\"uuid\":\"f3c21808-e34e-4785-8275-0070ba5b450f\"}],\"packageUris\":[\"http://schema.mathworks.com/mf0/Connector/R2020b\"],\"version\":\"1.0\"}"
      mask Display: disp('x')
  multb4_3 : Subsystem  AncestorBlock=My_FI_Operations/multb4_
      settings: LibrarySourceBlock=My_FI_Operations/multb4_  PortSchema="{\"entries\":[{\"content\":{\"sides\":[{\"content\":{\"connectorIds\":[\"In1\"]},\"type\":\"ConnectorPlacement.EquallySpacedRectSide\",\"uuid\":\"20461ecc-945a-453b-bec8-f18bcbd4d7ca\"},{\"content\":{\"connectorIds\":[],\"side\":\"RIGHT\"},\"type\":\"ConnectorPlacement.EquallySpacedRectSide\",\"uuid\":\"a806ae65-26a1-4387-823f-a90265b6c751\"},{\"content\":{\"connectorIds\":[\"In2\"],\"side\":\"TOP\"},\"type\":\"ConnectorPlacement.EquallySpacedRectSide\",\"uuid\":\"faa34e1a-fdc6-4b39-b604-acf00955d353\"},{\"content\":{\"connectorIds\":[\"Out1\"],\"side\":\"BOTTOM\"},\"type\":\"ConnectorPlacement.EquallySpacedRectSide\",\"uuid\":\"234e609c-6b95-41af-91dd-8a06091f2e10\"}]},\"type\":\"ConnectorPlacement.EquallySpacedConnector\",\"uuid\":\"f3c21808-e34e-4785-8275-0070ba5b450f\"}],\"packageUris\":[\"http://schema.mathworks.com/mf0/Connector/R2020b\"],\"version\":\"1.0\"}"
      mask Display: disp('x')
  multb6_1 : Subsystem  AncestorBlock=My_FI_Operations/multb6_
      settings: LibrarySourceBlock=My_FI_Operations/multb6_  PortSchema="{\"entries\":[{\"content\":{\"sides\":[{\"content\":{\"connectorIds\":[\"In1\"]},\"type\":\"ConnectorPlacement.EquallySpacedRectSide\",\"uuid\":\"20461ecc-945a-453b-bec8-f18bcbd4d7ca\"},{\"content\":{\"connectorIds\":[],\"side\":\"RIGHT\"},\"type\":\"ConnectorPlacement.EquallySpacedRectSide\",\"uuid\":\"a806ae65-26a1-4387-823f-a90265b6c751\"},{\"content\":{\"connectorIds\":[\"In2\"],\"side\":\"TOP\"},\"type\":\"ConnectorPlacement.EquallySpacedRectSide\",\"uuid\":\"faa34e1a-fdc6-4b39-b604-acf00955d353\"},{\"content\":{\"connectorIds\":[\"Out1\"],\"side\":\"BOTTOM\"},\"type\":\"ConnectorPlacement.EquallySpacedRectSide\",\"uuid\":\"31f2fa17-ae8c-4166-97ac-b63529612348\"}]},\"type\":\"ConnectorPlacement.EquallySpacedConnector\",\"uuid\":\"f3c21808-e34e-4785-8275-0070ba5b450f\"}],\"packageUris\":[\"http://schema.mathworks.com/mf0/Connector/R2020b\"],\"version\":\"1.0\"}"
      mask Display: disp('x')
  multb6_2 : Subsystem  AncestorBlock=My_FI_Operations/multb6_
      settings: LibrarySourceBlock=My_FI_Operations/multb6_  PortSchema="{\"entries\":[{\"content\":{\"sides\":[{\"content\":{\"connectorIds\":[\"In1\"]},\"type\":\"ConnectorPlacement.EquallySpacedRectSide\",\"uuid\":\"20461ecc-945a-453b-bec8-f18bcbd4d7ca\"},{\"content\":{\"connectorIds\":[],\"side\":\"RIGHT\"},\"type\":\"ConnectorPlacement.EquallySpacedRectSide\",\"uuid\":\"a806ae65-26a1-4387-823f-a90265b6c751\"},{\"content\":{\"connectorIds\":[\"In2\"],\"side\":\"TOP\"},\"type\":\"ConnectorPlacement.EquallySpacedRectSide\",\"uuid\":\"faa34e1a-fdc6-4b39-b604-acf00955d353\"},{\"content\":{\"connectorIds\":[\"Out1\"],\"side\":\"BOTTOM\"},\"type\":\"ConnectorPlacement.EquallySpacedRectSide\",\"uuid\":\"31f2fa17-ae8c-4166-97ac-b63529612348\"}]},\"type\":\"ConnectorPlacement.EquallySpacedConnector\",\"uuid\":\"f3c21808-e34e-4785-8275-0070ba5b450f\"}],\"packageUris\":[\"http://schema.mathworks.com/mf0/Connector/R2020b\"],\"version\":\"1.0\"}"
      mask Display: disp('x')
  multb6_3 : Subsystem  AncestorBlock=My_FI_Operations/multb6_
      settings: LibrarySourceBlock=My_FI_Operations/multb6_  PortSchema="{\"entries\":[{\"content\":{\"sides\":[{\"content\":{\"connectorIds\":[\"In1\"]},\"type\":\"ConnectorPlacement.EquallySpacedRectSide\",\"uuid\":\"20461ecc-945a-453b-bec8-f18bcbd4d7ca\"},{\"content\":{\"connectorIds\":[],\"side\":\"RIGHT\"},\"type\":\"ConnectorPlacement.EquallySpacedRectSide\",\"uuid\":\"a806ae65-26a1-4387-823f-a90265b6c751\"},{\"content\":{\"connectorIds\":[\"In2\"],\"side\":\"TOP\"},\"type\":\"ConnectorPlacement.EquallySpacedRectSide\",\"uuid\":\"faa34e1a-fdc6-4b39-b604-acf00955d353\"},{\"content\":{\"connectorIds\":[\"Out1\"],\"side\":\"BOTTOM\"},\"type\":\"ConnectorPlacement.EquallySpacedRectSide\",\"uuid\":\"31f2fa17-ae8c-4166-97ac-b63529612348\"}]},\"type\":\"ConnectorPlacement.EquallySpacedConnector\",\"uuid\":\"f3c21808-e34e-4785-8275-0070ba5b450f\"}],\"packageUris\":[\"http://schema.mathworks.com/mf0/Connector/R2020b\"],\"version\":\"1.0\"}"
      mask Display: disp('x')
  multb8_1 : Subsystem  AncestorBlock=My_FI_Operations/multb8_
      settings: LibrarySourceBlock=My_FI_Operations/multb8_  PortSchema="{\"entries\":[{\"content\":{\"sides\":[{\"content\":{\"connectorIds\":[\"In1\"]},\"type\":\"ConnectorPlacement.EquallySpacedRectSide\",\"uuid\":\"20461ecc-945a-453b-bec8-f18bcbd4d7ca\"},{\"content\":{\"connectorIds\":[],\"side\":\"RIGHT\"},\"type\":\"ConnectorPlacement.EquallySpacedRectSide\",\"uuid\":\"a806ae65-26a1-4387-823f-a90265b6c751\"},{\"content\":{\"connectorIds\":[\"In2\"],\"side\":\"TOP\"},\"type\":\"ConnectorPlacement.EquallySpacedRectSide\",\"uuid\":\"faa34e1a-fdc6-4b39-b604-acf00955d353\"},{\"content\":{\"connectorIds\":[\"Out1\"],\"side\":\"BOTTOM\"},\"type\":\"ConnectorPlacement.EquallySpacedRectSide\",\"uuid\":\"456c6a3b-895e-40a3-a775-e7e1c8929b79\"}]},\"type\":\"ConnectorPlacement.EquallySpacedConnector\",\"uuid\":\"f3c21808-e34e-4785-8275-0070ba5b450f\"}],\"packageUris\":[\"http://schema.mathworks.com/mf0/Connector/R2020b\"],\"version\":\"1.0\"}"
      mask Display: disp('x')
  multb8_2 : Subsystem  AncestorBlock=My_FI_Operations/multb8_
      settings: LibrarySourceBlock=My_FI_Operations/multb8_  PortSchema="{\"entries\":[{\"content\":{\"sides\":[{\"content\":{\"connectorIds\":[\"In1\"]},\"type\":\"ConnectorPlacement.EquallySpacedRectSide\",\"uuid\":\"20461ecc-945a-453b-bec8-f18bcbd4d7ca\"},{\"content\":{\"connectorIds\":[],\"side\":\"RIGHT\"},\"type\":\"ConnectorPlacement.EquallySpacedRectSide\",\"uuid\":\"a806ae65-26a1-4387-823f-a90265b6c751\"},{\"content\":{\"connectorIds\":[\"In2\"],\"side\":\"TOP\"},\"type\":\"ConnectorPlacement.EquallySpacedRectSide\",\"uuid\":\"faa34e1a-fdc6-4b39-b604-acf00955d353\"},{\"content\":{\"connectorIds\":[\"Out1\"],\"side\":\"BOTTOM\"},\"type\":\"ConnectorPlacement.EquallySpacedRectSide\",\"uuid\":\"456c6a3b-895e-40a3-a775-e7e1c8929b79\"}]},\"type\":\"ConnectorPlacement.EquallySpacedConnector\",\"uuid\":\"f3c21808-e34e-4785-8275-0070ba5b450f\"}],\"packageUris\":[\"http://schema.mathworks.com/mf0/Connector/R2020b\"],\"version\":\"1.0\"}"
      mask Display: disp('x')
  multb8_3 : Subsystem  AncestorBlock=My_FI_Operations/multb8_
      settings: LibrarySourceBlock=My_FI_Operations/multb8_  PortSchema="{\"entries\":[{\"content\":{\"sides\":[{\"content\":{\"connectorIds\":[\"In1\"]},\"type\":\"ConnectorPlacement.EquallySpacedRectSide\",\"uuid\":\"20461ecc-945a-453b-bec8-f18bcbd4d7ca\"},{\"content\":{\"connectorIds\":[],\"side\":\"RIGHT\"},\"type\":\"ConnectorPlacement.EquallySpacedRectSide\",\"uuid\":\"a806ae65-26a1-4387-823f-a90265b6c751\"},{\"content\":{\"connectorIds\":[\"In2\"],\"side\":\"TOP\"},\"type\":\"ConnectorPlacement.EquallySpacedRectSide\",\"uuid\":\"faa34e1a-fdc6-4b39-b604-acf00955d353\"},{\"content\":{\"connectorIds\":[\"Out1\"],\"side\":\"BOTTOM\"},\"type\":\"ConnectorPlacement.EquallySpacedRectSide\",\"uuid\":\"456c6a3b-895e-40a3-a775-e7e1c8929b79\"}]},\"type\":\"ConnectorPlacement.EquallySpacedConnector\",\"uuid\":\"f3c21808-e34e-4785-8275-0070ba5b450f\"}],\"packageUris\":[\"http://schema.mathworks.com/mf0/Connector/R2020b\"],\"version\":\"1.0\"}"
      mask Display: disp('x')
  suma2_1 : Subsystem  AncestorBlock=My_FI_Operations/suma2_
      settings: LibrarySourceBlock=My_FI_Operations/suma2_  PortSchema="{\"entries\":[{\"content\":{\"sides\":[{\"content\":{\"connectorIds\":[\"Out1\"]},\"type\":\"ConnectorPlacement.EquallySpacedRectSide\",\"uuid\":\"423828e0-6700-4575-ac06-a5fb7cb5569f\"},{\"content\":{\"connectorIds\":[\"In2\"],\"side\":\"RIGHT\"},\"type\":\"ConnectorPlacement.EquallySpacedRectSide\",\"uuid\":\"a42db842-eb55-44f2-8f04-0144bc45d908\"},{\"content\":{\"connectorIds\":[\"In1\"],\"side\":\"TOP\"},\"type\":\"ConnectorPlacement.EquallySpacedRectSide\",\"uuid\":\"eef5137d-31f0-46b4-a53b-5aa31464a7f9\"}]},\"type\":\"ConnectorPlacement.EquallySpacedConnector\",\"uuid\":\"7dd7fe03-b221-4701-a7b2-6552f08320da\"}],\"packageUris\":[\"http://schema.mathworks.com/mf0/Connector/R2020b\"],\"version\":\"1.0\"}"
      mask Display: disp('+')
  suma2_2 : Subsystem  AncestorBlock=My_FI_Operations/suma2_
      settings: LibrarySourceBlock=My_FI_Operations/suma2_  PortSchema="{\"entries\":[{\"content\":{\"sides\":[{\"content\":{\"connectorIds\":[\"Out1\"]},\"type\":\"ConnectorPlacement.EquallySpacedRectSide\",\"uuid\":\"423828e0-6700-4575-ac06-a5fb7cb5569f\"},{\"content\":{\"connectorIds\":[\"In2\"],\"side\":\"RIGHT\"},\"type\":\"ConnectorPlacement.EquallySpacedRectSide\",\"uuid\":\"a42db842-eb55-44f2-8f04-0144bc45d908\"},{\"content\":{\"connectorIds\":[\"In1\"],\"side\":\"TOP\"},\"type\":\"ConnectorPlacement.EquallySpacedRectSide\",\"uuid\":\"eef5137d-31f0-46b4-a53b-5aa31464a7f9\"}]},\"type\":\"ConnectorPlacement.EquallySpacedConnector\",\"uuid\":\"7dd7fe03-b221-4701-a7b2-6552f08320da\"}],\"packageUris\":[\"http://schema.mathworks.com/mf0/Connector/R2020b\"],\"version\":\"1.0\"}"
      mask Display: disp('+')
  suma2_3 : Subsystem  AncestorBlock=My_FI_Operations/suma2_
      settings: LibrarySourceBlock=My_FI_Operations/suma2_  PortSchema="{\"entries\":[{\"content\":{\"sides\":[{\"content\":{\"connectorIds\":[\"Out1\"]},\"type\":\"ConnectorPlacement.EquallySpacedRectSide\",\"uuid\":\"423828e0-6700-4575-ac06-a5fb7cb5569f\"},{\"content\":{\"connectorIds\":[\"In2\"],\"side\":\"RIGHT\"},\"type\":\"ConnectorPlacement.EquallySpacedRectSide\",\"uuid\":\"a42db842-eb55-44f2-8f04-0144bc45d908\"},{\"content\":{\"connectorIds\":[\"In1\"],\"side\":\"TOP\"},\"type\":\"ConnectorPlacement.EquallySpacedRectSide\",\"uuid\":\"eef5137d-31f0-46b4-a53b-5aa31464a7f9\"}]},\"type\":\"ConnectorPlacement.EquallySpacedConnector\",\"uuid\":\"7dd7fe03-b221-4701-a7b2-6552f08320da\"}],\"packageUris\":[\"http://schema.mathworks.com/mf0/Connector/R2020b\"],\"version\":\"1.0\"}"
      mask Display: disp('+')
  suma4_1 : Subsystem  AncestorBlock=My_FI_Operations/suma4_
      settings: LibrarySourceBlock=My_FI_Operations/suma4_  PortSchema="{\"entries\":[{\"content\":{\"sides\":[{\"content\":{\"connectorIds\":[\"Out1\"]},\"type\":\"ConnectorPlacement.EquallySpacedRectSide\",\"uuid\":\"423828e0-6700-4575-ac06-a5fb7cb5569f\"},{\"content\":{\"connectorIds\":[\"In2\"],\"side\":\"RIGHT\"},\"type\":\"ConnectorPlacement.EquallySpacedRectSide\",\"uuid\":\"a42db842-eb55-44f2-8f04-0144bc45d908\"},{\"content\":{\"connectorIds\":[\"In1\"],\"side\":\"TOP\"},\"type\":\"ConnectorPlacement.EquallySpacedRectSide\",\"uuid\":\"eef5137d-31f0-46b4-a53b-5aa31464a7f9\"}]},\"type\":\"ConnectorPlacement.EquallySpacedConnector\",\"uuid\":\"7dd7fe03-b221-4701-a7b2-6552f08320da\"}],\"packageUris\":[\"http://schema.mathworks.com/mf0/Connector/R2020b\"],\"version\":\"1.0\"}"
      mask Display: disp('+')
  suma4_2 : Subsystem  AncestorBlock=My_FI_Operations/suma4_
      settings: LibrarySourceBlock=My_FI_Operations/suma4_  PortSchema="{\"entries\":[{\"content\":{\"sides\":[{\"content\":{\"connectorIds\":[\"Out1\"]},\"type\":\"ConnectorPlacement.EquallySpacedRectSide\",\"uuid\":\"423828e0-6700-4575-ac06-a5fb7cb5569f\"},{\"content\":{\"connectorIds\":[\"In2\"],\"side\":\"RIGHT\"},\"type\":\"ConnectorPlacement.EquallySpacedRectSide\",\"uuid\":\"a42db842-eb55-44f2-8f04-0144bc45d908\"},{\"content\":{\"connectorIds\":[\"In1\"],\"side\":\"TOP\"},\"type\":\"ConnectorPlacement.EquallySpacedRectSide\",\"uuid\":\"eef5137d-31f0-46b4-a53b-5aa31464a7f9\"}]},\"type\":\"ConnectorPlacement.EquallySpacedConnector\",\"uuid\":\"7dd7fe03-b221-4701-a7b2-6552f08320da\"}],\"packageUris\":[\"http://schema.mathworks.com/mf0/Connector/R2020b\"],\"version\":\"1.0\"}"
      mask Display: disp('+')
  suma4_3 : Subsystem  AncestorBlock=My_FI_Operations/suma4_
      settings: LibrarySourceBlock=My_FI_Operations/suma4_  PortSchema="{\"entries\":[{\"content\":{\"sides\":[{\"content\":{\"connectorIds\":[\"Out1\"]},\"type\":\"ConnectorPlacement.EquallySpacedRectSide\",\"uuid\":\"423828e0-6700-4575-ac06-a5fb7cb5569f\"},{\"content\":{\"connectorIds\":[\"In2\"],\"side\":\"RIGHT\"},\"type\":\"ConnectorPlacement.EquallySpacedRectSide\",\"uuid\":\"a42db842-eb55-44f2-8f04-0144bc45d908\"},{\"content\":{\"connectorIds\":[\"In1\"],\"side\":\"TOP\"},\"type\":\"ConnectorPlacement.EquallySpacedRectSide\",\"uuid\":\"eef5137d-31f0-46b4-a53b-5aa31464a7f9\"}]},\"type\":\"ConnectorPlacement.EquallySpacedConnector\",\"uuid\":\"7dd7fe03-b221-4701-a7b2-6552f08320da\"}],\"packageUris\":[\"http://schema.mathworks.com/mf0/Connector/R2020b\"],\"version\":\"1.0\"}"
      mask Display: disp('+')
  suma6_1 : Subsystem  AncestorBlock=My_FI_Operations/suma6_
      settings: LibrarySourceBlock=My_FI_Operations/suma6_  PortSchema="{\"entries\":[{\"content\":{\"sides\":[{\"content\":{\"connectorIds\":[\"Out1\"]},\"type\":\"ConnectorPlacement.EquallySpacedRectSide\",\"uuid\":\"423828e0-6700-4575-ac06-a5fb7cb5569f\"},{\"content\":{\"connectorIds\":[\"In2\"],\"side\":\"RIGHT\"},\"type\":\"ConnectorPlacement.EquallySpacedRectSide\",\"uuid\":\"a42db842-eb55-44f2-8f04-0144bc45d908\"},{\"content\":{\"connectorIds\":[\"In1\"],\"side\":\"TOP\"},\"type\":\"ConnectorPlacement.EquallySpacedRectSide\",\"uuid\":\"eef5137d-31f0-46b4-a53b-5aa31464a7f9\"}]},\"type\":\"ConnectorPlacement.EquallySpacedConnector\",\"uuid\":\"7dd7fe03-b221-4701-a7b2-6552f08320da\"}],\"packageUris\":[\"http://schema.mathworks.com/mf0/Connector/R2020b\"],\"version\":\"1.0\"}"
      mask Display: disp('+')
  suma6_2 : Subsystem  AncestorBlock=My_FI_Operations/suma6_
      settings: LibrarySourceBlock=My_FI_Operations/suma6_  PortSchema="{\"entries\":[{\"content\":{\"sides\":[{\"content\":{\"connectorIds\":[\"Out1\"]},\"type\":\"ConnectorPlacement.EquallySpacedRectSide\",\"uuid\":\"423828e0-6700-4575-ac06-a5fb7cb5569f\"},{\"content\":{\"connectorIds\":[\"In2\"],\"side\":\"RIGHT\"},\"type\":\"ConnectorPlacement.EquallySpacedRectSide\",\"uuid\":\"a42db842-eb55-44f2-8f04-0144bc45d908\"},{\"content\":{\"connectorIds\":[\"In1\"],\"side\":\"TOP\"},\"type\":\"ConnectorPlacement.EquallySpacedRectSide\",\"uuid\":\"eef5137d-31f0-46b4-a53b-5aa31464a7f9\"}]},\"type\":\"ConnectorPlacement.EquallySpacedConnector\",\"uuid\":\"7dd7fe03-b221-4701-a7b2-6552f08320da\"}],\"packageUris\":[\"http://schema.mathworks.com/mf0/Connector/R2020b\"],\"version\":\"1.0\"}"
      mask Display: disp('+')
  suma6_3 : Subsystem  AncestorBlock=My_FI_Operations/suma6_
      settings: LibrarySourceBlock=My_FI_Operations/suma6_  PortSchema="{\"entries\":[{\"content\":{\"sides\":[{\"content\":{\"connectorIds\":[\"Out1\"]},\"type\":\"ConnectorPlacement.EquallySpacedRectSide\",\"uuid\":\"423828e0-6700-4575-ac06-a5fb7cb5569f\"},{\"content\":{\"connectorIds\":[\"In2\"],\"side\":\"RIGHT\"},\"type\":\"ConnectorPlacement.EquallySpacedRectSide\",\"uuid\":\"a42db842-eb55-44f2-8f04-0144bc45d908\"},{\"content\":{\"connectorIds\":[\"In1\"],\"side\":\"TOP\"},\"type\":\"ConnectorPlacement.EquallySpacedRectSide\",\"uuid\":\"eef5137d-31f0-46b4-a53b-5aa31464a7f9\"}]},\"type\":\"ConnectorPlacement.EquallySpacedConnector\",\"uuid\":\"7dd7fe03-b221-4701-a7b2-6552f08320da\"}],\"packageUris\":[\"http://schema.mathworks.com/mf0/Connector/R2020b\"],\"version\":\"1.0\"}"
      mask Display: disp('+')
  sumb10_1 : Subsystem  AncestorBlock=My_FI_Operations/sumb10_
      settings: LibrarySourceBlock=My_FI_Operations/sumb10_  PortSchema="{\"entries\":[{\"content\":{\"sides\":[{\"content\":{\"connectorIds\":[\"In1\"]},\"type\":\"ConnectorPlacement.EquallySpacedRectSide\",\"uuid\":\"20461ecc-945a-453b-bec8-f18bcbd4d7ca\"},{\"content\":{\"connectorIds\":[\"Out1\"],\"side\":\"RIGHT\"},\"type\":\"ConnectorPlacement.EquallySpacedRectSide\",\"uuid\":\"a806ae65-26a1-4387-823f-a90265b6c751\"},{\"content\":{\"connectorIds\":[\"In2\"],\"side\":\"TOP\"},\"type\":\"ConnectorPlacement.EquallySpacedRectSide\",\"uuid\":\"faa34e1a-fdc6-4b39-b604-acf00955d353\"}]},\"type\":\"ConnectorPlacement.EquallySpacedConnector\",\"uuid\":\"f3c21808-e34e-4785-8275-0070ba5b450f\"}],\"packageUris\":[\"http://schema.mathworks.com/mf0/Connector/R2020b\"],\"version\":\"1.0\"}"
      mask Display: disp('+')
  sumb10_2 : Subsystem  AncestorBlock=My_FI_Operations/sumb10_
      settings: LibrarySourceBlock=My_FI_Operations/sumb10_  PortSchema="{\"entries\":[{\"content\":{\"sides\":[{\"content\":{\"connectorIds\":[\"In1\"]},\"type\":\"ConnectorPlacement.EquallySpacedRectSide\",\"uuid\":\"20461ecc-945a-453b-bec8-f18bcbd4d7ca\"},{\"content\":{\"connectorIds\":[\"Out1\"],\"side\":\"RIGHT\"},\"type\":\"ConnectorPlacement.EquallySpacedRectSide\",\"uuid\":\"a806ae65-26a1-4387-823f-a90265b6c751\"},{\"content\":{\"connectorIds\":[\"In2\"],\"side\":\"TOP\"},\"type\":\"ConnectorPlacement.EquallySpacedRectSide\",\"uuid\":\"faa34e1a-fdc6-4b39-b604-acf00955d353\"}]},\"type\":\"ConnectorPlacement.EquallySpacedConnector\",\"uuid\":\"f3c21808-e34e-4785-8275-0070ba5b450f\"}],\"packageUris\":[\"http://schema.mathworks.com/mf0/Connector/R2020b\"],\"version\":\"1.0\"}"
      mask Display: disp('+')
  sumb10_3 : Subsystem  AncestorBlock=My_FI_Operations/sumb10_
      settings: LibrarySourceBlock=My_FI_Operations/sumb10_  PortSchema="{\"entries\":[{\"content\":{\"sides\":[{\"content\":{\"connectorIds\":[\"In1\"]},\"type\":\"ConnectorPlacement.EquallySpacedRectSide\",\"uuid\":\"20461ecc-945a-453b-bec8-f18bcbd4d7ca\"},{\"content\":{\"connectorIds\":[\"Out1\"],\"side\":\"RIGHT\"},\"type\":\"ConnectorPlacement.EquallySpacedRectSide\",\"uuid\":\"a806ae65-26a1-4387-823f-a90265b6c751\"},{\"content\":{\"connectorIds\":[\"In2\"],\"side\":\"TOP\"},\"type\":\"ConnectorPlacement.EquallySpacedRectSide\",\"uuid\":\"faa34e1a-fdc6-4b39-b604-acf00955d353\"}]},\"type\":\"ConnectorPlacement.EquallySpacedConnector\",\"uuid\":\"f3c21808-e34e-4785-8275-0070ba5b450f\"}],\"packageUris\":[\"http://schema.mathworks.com/mf0/Connector/R2020b\"],\"version\":\"1.0\"}"
      mask Display: disp('+')
  sumb12_1 : Subsystem  AncestorBlock=My_FI_Operations/sumb12_
      settings: LibrarySourceBlock=My_FI_Operations/sumb12_  PortSchema="{\"entries\":[{\"content\":{\"sides\":[{\"content\":{\"connectorIds\":[\"In1\"]},\"type\":\"ConnectorPlacement.EquallySpacedRectSide\",\"uuid\":\"20461ecc-945a-453b-bec8-f18bcbd4d7ca\"},{\"content\":{\"connectorIds\":[\"Out1\"],\"side\":\"RIGHT\"},\"type\":\"ConnectorPlacement.EquallySpacedRectSide\",\"uuid\":\"a806ae65-26a1-4387-823f-a90265b6c751\"},{\"content\":{\"connectorIds\":[\"In2\"],\"side\":\"TOP\"},\"type\":\"ConnectorPlacement.EquallySpacedRectSide\",\"uuid\":\"faa34e1a-fdc6-4b39-b604-acf00955d353\"}]},\"type\":\"ConnectorPlacement.EquallySpacedConnector\",\"uuid\":\"f3c21808-e34e-4785-8275-0070ba5b450f\"}],\"packageUris\":[\"http://schema.mathworks.com/mf0/Connector/R2020b\"],\"version\":\"1.0\"}"
      mask Display: disp('+')
  sumb12_2 : Subsystem  AncestorBlock=My_FI_Operations/sumb12_
      settings: LibrarySourceBlock=My_FI_Operations/sumb12_  PortSchema="{\"entries\":[{\"content\":{\"sides\":[{\"content\":{\"connectorIds\":[\"In1\"]},\"type\":\"ConnectorPlacement.EquallySpacedRectSide\",\"uuid\":\"20461ecc-945a-453b-bec8-f18bcbd4d7ca\"},{\"content\":{\"connectorIds\":[\"Out1\"],\"side\":\"RIGHT\"},\"type\":\"ConnectorPlacement.EquallySpacedRectSide\",\"uuid\":\"a806ae65-26a1-4387-823f-a90265b6c751\"},{\"content\":{\"connectorIds\":[\"In2\"],\"side\":\"TOP\"},\"type\":\"ConnectorPlacement.EquallySpacedRectSide\",\"uuid\":\"faa34e1a-fdc6-4b39-b604-acf00955d353\"}]},\"type\":\"ConnectorPlacement.EquallySpacedConnector\",\"uuid\":\"f3c21808-e34e-4785-8275-0070ba5b450f\"}],\"packageUris\":[\"http://schema.mathworks.com/mf0/Connector/R2020b\"],\"version\":\"1.0\"}"
      mask Display: disp('+')
  sumb12_3 : Subsystem  AncestorBlock=My_FI_Operations/sumb12_
      settings: LibrarySourceBlock=My_FI_Operations/sumb12_  PortSchema="{\"entries\":[{\"content\":{\"sides\":[{\"content\":{\"connectorIds\":[\"In1\"]},\"type\":\"ConnectorPlacement.EquallySpacedRectSide\",\"uuid\":\"20461ecc-945a-453b-bec8-f18bcbd4d7ca\"},{\"content\":{\"connectorIds\":[\"Out1\"],\"side\":\"RIGHT\"},\"type\":\"ConnectorPlacement.EquallySpacedRectSide\",\"uuid\":\"a806ae65-26a1-4387-823f-a90265b6c751\"},{\"content\":{\"connectorIds\":[\"In2\"],\"side\":\"TOP\"},\"type\":\"ConnectorPlacement.EquallySpacedRectSide\",\"uuid\":\"faa34e1a-fdc6-4b39-b604-acf00955d353\"}]},\"type\":\"ConnectorPlacement.EquallySpacedConnector\",\"uuid\":\"f3c21808-e34e-4785-8275-0070ba5b450f\"}],\"packageUris\":[\"http://schema.mathworks.com/mf0/Connector/R2020b\"],\"version\":\"1.0\"}"
      mask Display: disp('+')
  sumb2_1 : Subsystem  AncestorBlock=My_FI_Operations/sumb2_
      settings: LibrarySourceBlock=My_FI_Operations/sumb2_  PortSchema="{\"entries\":[{\"content\":{\"sides\":[{\"content\":{\"connectorIds\":[\"In1\"]},\"type\":\"ConnectorPlacement.EquallySpacedRectSide\",\"uuid\":\"20461ecc-945a-453b-bec8-f18bcbd4d7ca\"},{\"content\":{\"connectorIds\":[\"Out1\"],\"side\":\"RIGHT\"},\"type\":\"ConnectorPlacement.EquallySpacedRectSide\",\"uuid\":\"a806ae65-26a1-4387-823f-a90265b6c751\"},{\"content\":{\"connectorIds\":[\"In2\"],\"side\":\"TOP\"},\"type\":\"ConnectorPlacement.EquallySpacedRectSide\",\"uuid\":\"faa34e1a-fdc6-4b39-b604-acf00955d353\"}]},\"type\":\"ConnectorPlacement.EquallySpacedConnector\",\"uuid\":\"f3c21808-e34e-4785-8275-0070ba5b450f\"}],\"packageUris\":[\"http://schema.mathworks.com/mf0/Connector/R2020b\"],\"version\":\"1.0\"}"
      mask Display: disp('+')
  sumb2_2 : Subsystem  AncestorBlock=My_FI_Operations/sumb2_
      settings: LibrarySourceBlock=My_FI_Operations/sumb2_  PortSchema="{\"entries\":[{\"content\":{\"sides\":[{\"content\":{\"connectorIds\":[\"In1\"]},\"type\":\"ConnectorPlacement.EquallySpacedRectSide\",\"uuid\":\"20461ecc-945a-453b-bec8-f18bcbd4d7ca\"},{\"content\":{\"connectorIds\":[\"Out1\"],\"side\":\"RIGHT\"},\"type\":\"ConnectorPlacement.EquallySpacedRectSide\",\"uuid\":\"a806ae65-26a1-4387-823f-a90265b6c751\"},{\"content\":{\"connectorIds\":[\"In2\"],\"side\":\"TOP\"},\"type\":\"ConnectorPlacement.EquallySpacedRectSide\",\"uuid\":\"faa34e1a-fdc6-4b39-b604-acf00955d353\"}]},\"type\":\"ConnectorPlacement.EquallySpacedConnector\",\"uuid\":\"f3c21808-e34e-4785-8275-0070ba5b450f\"}],\"packageUris\":[\"http://schema.mathworks.com/mf0/Connector/R2020b\"],\"version\":\"1.0\"}"
      mask Display: disp('+')
  sumb2_3 : Subsystem  AncestorBlock=My_FI_Operations/sumb2_
      settings: LibrarySourceBlock=My_FI_Operations/sumb2_  PortSchema="{\"entries\":[{\"content\":{\"sides\":[{\"content\":{\"connectorIds\":[\"In1\"]},\"type\":\"ConnectorPlacement.EquallySpacedRectSide\",\"uuid\":\"20461ecc-945a-453b-bec8-f18bcbd4d7ca\"},{\"content\":{\"connectorIds\":[\"Out1\"],\"side\":\"RIGHT\"},\"type\":\"ConnectorPlacement.EquallySpacedRectSide\",\"uuid\":\"a806ae65-26a1-4387-823f-a90265b6c751\"},{\"content\":{\"connectorIds\":[\"In2\"],\"side\":\"TOP\"},\"type\":\"ConnectorPlacement.EquallySpacedRectSide\",\"uuid\":\"faa34e1a-fdc6-4b39-b604-acf00955d353\"}]},\"type\":\"ConnectorPlacement.EquallySpacedConnector\",\"uuid\":\"f3c21808-e34e-4785-8275-0070ba5b450f\"}],\"packageUris\":[\"http://schema.mathworks.com/mf0/Connector/R2020b\"],\"version\":\"1.0\"}"
      mask Display: disp('+')
  sumb4_1 : Subsystem  AncestorBlock=My_FI_Operations/sumb4_
      settings: LibrarySourceBlock=My_FI_Operations/sumb4_  PortSchema="{\"entries\":[{\"content\":{\"sides\":[{\"content\":{\"connectorIds\":[\"In1\"]},\"type\":\"ConnectorPlacement.EquallySpacedRectSide\",\"uuid\":\"20461ecc-945a-453b-bec8-f18bcbd4d7ca\"},{\"content\":{\"connectorIds\":[\"Out1\"],\"side\":\"RIGHT\"},\"type\":\"ConnectorPlacement.EquallySpacedRectSide\",\"uuid\":\"a806ae65-26a1-4387-823f-a90265b6c751\"},{\"content\":{\"connectorIds\":[\"In2\"],\"side\":\"TOP\"},\"type\":\"ConnectorPlacement.EquallySpacedRectSide\",\"uuid\":\"faa34e1a-fdc6-4b39-b604-acf00955d353\"}]},\"type\":\"ConnectorPlacement.EquallySpacedConnector\",\"uuid\":\"f3c21808-e34e-4785-8275-0070ba5b450f\"}],\"packageUris\":[\"http://schema.mathworks.com/mf0/Connector/R2020b\"],\"version\":\"1.0\"}"
      mask Display: disp('+')
  sumb4_2 : Subsystem  AncestorBlock=My_FI_Operations/sumb4_
      settings: LibrarySourceBlock=My_FI_Operations/sumb4_  PortSchema="{\"entries\":[{\"content\":{\"sides\":[{\"content\":{\"connectorIds\":[\"In1\"]},\"type\":\"ConnectorPlacement.EquallySpacedRectSide\",\"uuid\":\"20461ecc-945a-453b-bec8-f18bcbd4d7ca\"},{\"content\":{\"connectorIds\":[\"Out1\"],\"side\":\"RIGHT\"},\"type\":\"ConnectorPlacement.EquallySpacedRectSide\",\"uuid\":\"a806ae65-26a1-4387-823f-a90265b6c751\"},{\"content\":{\"connectorIds\":[\"In2\"],\"side\":\"TOP\"},\"type\":\"ConnectorPlacement.EquallySpacedRectSide\",\"uuid\":\"faa34e1a-fdc6-4b39-b604-acf00955d353\"}]},\"type\":\"ConnectorPlacement.EquallySpacedConnector\",\"uuid\":\"f3c21808-e34e-4785-8275-0070ba5b450f\"}],\"packageUris\":[\"http://schema.mathworks.com/mf0/Connector/R2020b\"],\"version\":\"1.0\"}"
      mask Display: disp('+')
  sumb4_3 : Subsystem  AncestorBlock=My_FI_Operations/sumb4_
      settings: LibrarySourceBlock=My_FI_Operations/sumb4_  PortSchema="{\"entries\":[{\"content\":{\"sides\":[{\"content\":{\"connectorIds\":[\"In1\"]},\"type\":\"ConnectorPlacement.EquallySpacedRectSide\",\"uuid\":\"20461ecc-945a-453b-bec8-f18bcbd4d7ca\"},{\"content\":{\"connectorIds\":[\"Out1\"],\"side\":\"RIGHT\"},\"type\":\"ConnectorPlacement.EquallySpacedRectSide\",\"uuid\":\"a806ae65-26a1-4387-823f-a90265b6c751\"},{\"content\":{\"connectorIds\":[\"In2\"],\"side\":\"TOP\"},\"type\":\"ConnectorPlacement.EquallySpacedRectSide\",\"uuid\":\"faa34e1a-fdc6-4b39-b604-acf00955d353\"}]},\"type\":\"ConnectorPlacement.EquallySpacedConnector\",\"uuid\":\"f3c21808-e34e-4785-8275-0070ba5b450f\"}],\"packageUris\":[\"http://schema.mathworks.com/mf0/Connector/R2020b\"],\"version\":\"1.0\"}"
      mask Display: disp('+')
  sumb6_1 : Subsystem  AncestorBlock=My_FI_Operations/sumb6_
      settings: LibrarySourceBlock=My_FI_Operations/sumb6_  PortSchema="{\"entries\":[{\"content\":{\"sides\":[{\"content\":{\"connectorIds\":[\"In1\"]},\"type\":\"ConnectorPlacement.EquallySpacedRectSide\",\"uuid\":\"20461ecc-945a-453b-bec8-f18bcbd4d7ca\"},{\"content\":{\"connectorIds\":[\"Out1\"],\"side\":\"RIGHT\"},\"type\":\"ConnectorPlacement.EquallySpacedRectSide\",\"uuid\":\"a806ae65-26a1-4387-823f-a90265b6c751\"},{\"content\":{\"connectorIds\":[\"In2\"],\"side\":\"TOP\"},\"type\":\"ConnectorPlacement.EquallySpacedRectSide\",\"uuid\":\"faa34e1a-fdc6-4b39-b604-acf00955d353\"}]},\"type\":\"ConnectorPlacement.EquallySpacedConnector\",\"uuid\":\"f3c21808-e34e-4785-8275-0070ba5b450f\"}],\"packageUris\":[\"http://schema.mathworks.com/mf0/Connector/R2020b\"],\"version\":\"1.0\"}"
      mask Display: disp('+')
  sumb6_2 : Subsystem  AncestorBlock=My_FI_Operations/sumb6_
      settings: LibrarySourceBlock=My_FI_Operations/sumb6_  PortSchema="{\"entries\":[{\"content\":{\"sides\":[{\"content\":{\"connectorIds\":[\"In1\"]},\"type\":\"ConnectorPlacement.EquallySpacedRectSide\",\"uuid\":\"20461ecc-945a-453b-bec8-f18bcbd4d7ca\"},{\"content\":{\"connectorIds\":[\"Out1\"],\"side\":\"RIGHT\"},\"type\":\"ConnectorPlacement.EquallySpacedRectSide\",\"uuid\":\"a806ae65-26a1-4387-823f-a90265b6c751\"},{\"content\":{\"connectorIds\":[\"In2\"],\"side\":\"TOP\"},\"type\":\"ConnectorPlacement.EquallySpacedRectSide\",\"uuid\":\"faa34e1a-fdc6-4b39-b604-acf00955d353\"}]},\"type\":\"ConnectorPlacement.EquallySpacedConnector\",\"uuid\":\"f3c21808-e34e-4785-8275-0070ba5b450f\"}],\"packageUris\":[\"http://schema.mathworks.com/mf0/Connector/R2020b\"],\"version\":\"1.0\"}"
      mask Display: disp('+')
  sumb6_3 : Subsystem  AncestorBlock=My_FI_Operations/sumb6_
      settings: LibrarySourceBlock=My_FI_Operations/sumb6_  PortSchema="{\"entries\":[{\"content\":{\"sides\":[{\"content\":{\"connectorIds\":[\"In1\"]},\"type\":\"ConnectorPlacement.EquallySpacedRectSide\",\"uuid\":\"20461ecc-945a-453b-bec8-f18bcbd4d7ca\"},{\"content\":{\"connectorIds\":[\"Out1\"],\"side\":\"RIGHT\"},\"type\":\"ConnectorPlacement.EquallySpacedRectSide\",\"uuid\":\"a806ae65-26a1-4387-823f-a90265b6c751\"},{\"content\":{\"connectorIds\":[\"In2\"],\"side\":\"TOP\"},\"type\":\"ConnectorPlacement.EquallySpacedRectSide\",\"uuid\":\"faa34e1a-fdc6-4b39-b604-acf00955d353\"}]},\"type\":\"ConnectorPlacement.EquallySpacedConnector\",\"uuid\":\"f3c21808-e34e-4785-8275-0070ba5b450f\"}],\"packageUris\":[\"http://schema.mathworks.com/mf0/Connector/R2020b\"],\"version\":\"1.0\"}"
      mask Display: disp('+')
  sumb8_1 : Subsystem  AncestorBlock=My_FI_Operations/sumb8_
      settings: LibrarySourceBlock=My_FI_Operations/sumb8_  PortSchema="{\"entries\":[{\"content\":{\"sides\":[{\"content\":{\"connectorIds\":[\"In1\"]},\"type\":\"ConnectorPlacement.EquallySpacedRectSide\",\"uuid\":\"20461ecc-945a-453b-bec8-f18bcbd4d7ca\"},{\"content\":{\"connectorIds\":[\"Out1\"],\"side\":\"RIGHT\"},\"type\":\"ConnectorPlacement.EquallySpacedRectSide\",\"uuid\":\"a806ae65-26a1-4387-823f-a90265b6c751\"},{\"content\":{\"connectorIds\":[\"In2\"],\"side\":\"TOP\"},\"type\":\"ConnectorPlacement.EquallySpacedRectSide\",\"uuid\":\"faa34e1a-fdc6-4b39-b604-acf00955d353\"}]},\"type\":\"ConnectorPlacement.EquallySpacedConnector\",\"uuid\":\"f3c21808-e34e-4785-8275-0070ba5b450f\"}],\"packageUris\":[\"http://schema.mathworks.com/mf0/Connector/R2020b\"],\"version\":\"1.0\"}"
      mask Display: disp('+')
  sumb8_2 : Subsystem  AncestorBlock=My_FI_Operations/sumb8_
      settings: LibrarySourceBlock=My_FI_Operations/sumb8_  PortSchema="{\"entries\":[{\"content\":{\"sides\":[{\"content\":{\"connectorIds\":[\"In1\"]},\"type\":\"ConnectorPlacement.EquallySpacedRectSide\",\"uuid\":\"20461ecc-945a-453b-bec8-f18bcbd4d7ca\"},{\"content\":{\"connectorIds\":[\"Out1\"],\"side\":\"RIGHT\"},\"type\":\"ConnectorPlacement.EquallySpacedRectSide\",\"uuid\":\"a806ae65-26a1-4387-823f-a90265b6c751\"},{\"content\":{\"connectorIds\":[\"In2\"],\"side\":\"TOP\"},\"type\":\"ConnectorPlacement.EquallySpacedRectSide\",\"uuid\":\"faa34e1a-fdc6-4b39-b604-acf00955d353\"}]},\"type\":\"ConnectorPlacement.EquallySpacedConnector\",\"uuid\":\"f3c21808-e34e-4785-8275-0070ba5b450f\"}],\"packageUris\":[\"http://schema.mathworks.com/mf0/Connector/R2020b\"],\"version\":\"1.0\"}"
      mask Display: disp('+')
  sumb8_3 : Subsystem  AncestorBlock=My_FI_Operations/sumb8_
      settings: LibrarySourceBlock=My_FI_Operations/sumb8_  PortSchema="{\"entries\":[{\"content\":{\"sides\":[{\"content\":{\"connectorIds\":[\"In1\"]},\"type\":\"ConnectorPlacement.EquallySpacedRectSide\",\"uuid\":\"20461ecc-945a-453b-bec8-f18bcbd4d7ca\"},{\"content\":{\"connectorIds\":[\"Out1\"],\"side\":\"RIGHT\"},\"type\":\"ConnectorPlacement.EquallySpacedRectSide\",\"uuid\":\"a806ae65-26a1-4387-823f-a90265b6c751\"},{\"content\":{\"connectorIds\":[\"In2\"],\"side\":\"TOP\"},\"type\":\"ConnectorPlacement.EquallySpacedRectSide\",\"uuid\":\"faa34e1a-fdc6-4b39-b604-acf00955d353\"}]},\"type\":\"ConnectorPlacement.EquallySpacedConnector\",\"uuid\":\"f3c21808-e34e-4785-8275-0070ba5b450f\"}],\"packageUris\":[\"http://schema.mathworks.com/mf0/Connector/R2020b\"],\"version\":\"1.0\"}"
      mask Display: disp('+')
  sumd-2 : Subsystem  AncestorBlock=My_FI_Operations/sumd-2
      settings: LibrarySourceBlock=My_FI_Operations/sumd-2  PortSchema="{\"entries\":[{\"content\":{\"sides\":[{\"content\":{\"connectorIds\":[]},\"type\":\"ConnectorPlacement.EquallySpacedRectSide\",\"uuid\":\"423828e0-6700-4575-ac06-a5fb7cb5569f\"},{\"content\":{\"connectorIds\":[\"In2\"],\"side\":\"RIGHT\"},\"type\":\"ConnectorPlacement.EquallySpacedRectSide\",\"uuid\":\"a42db842-eb55-44f2-8f04-0144bc45d908\"},{\"content\":{\"connectorIds\":[\"Out1\"],\"side\":\"TOP\"},\"type\":\"ConnectorPlacement.EquallySpacedRectSide\",\"uuid\":\"eef5137d-31f0-46b4-a53b-5aa31464a7f9\"},{\"content\":{\"connectorIds\":[\"In1\"],\"side\":\"BOTTOM\"},\"type\":\"ConnectorPlacement.EquallySpacedRectSide\",\"uuid\":\"0a29e77a-4bdf-45d0-8a25-1103c3446174\"}]},\"type\":\"ConnectorPlacement.EquallySpacedConnector\",\"uuid\":\"7dd7fe03-b221-4701-a7b2-6552f08320da\"}],\"packageUris\":[\"http://schema.mathworks.com/mf0/Connector/R2020b\"],\"version\":\"1.0\"}"
      mask Display: disp('+')
  sumd-3 : Subsystem  AncestorBlock=My_FI_Operations/sumd-3
      settings: LibrarySourceBlock=My_FI_Operations/sumd-3  PortSchema="{\"entries\":[{\"content\":{\"sides\":[{\"content\":{\"connectorIds\":[\"In1\"]},\"type\":\"ConnectorPlacement.EquallySpacedRectSide\",\"uuid\":\"423828e0-6700-4575-ac06-a5fb7cb5569f\"},{\"content\":{\"connectorIds\":[\"In2\"],\"side\":\"RIGHT\"},\"type\":\"ConnectorPlacement.EquallySpacedRectSide\",\"uuid\":\"a42db842-eb55-44f2-8f04-0144bc45d908\"},{\"content\":{\"connectorIds\":[\"Out1\"],\"side\":\"TOP\"},\"type\":\"ConnectorPlacement.EquallySpacedRectSide\",\"uuid\":\"eef5137d-31f0-46b4-a53b-5aa31464a7f9\"},{\"content\":{\"connectorIds\":[],\"side\":\"BOTTOM\"},\"type\":\"ConnectorPlacement.EquallySpacedRectSide\",\"uuid\":\"d67bc59d-e0b5-4328-b5c7-58ea1a954934\"}]},\"type\":\"ConnectorPlacement.EquallySpacedConnector\",\"uuid\":\"7dd7fe03-b221-4701-a7b2-6552f08320da\"}],\"packageUris\":[\"http://schema.mathworks.com/mf0/Connector/R2020b\"],\"version\":\"1.0\"}"
      mask Display: disp('+')
  sumd-4 : Subsystem  AncestorBlock=My_FI_Operations/sumd-4
      settings: LibrarySourceBlock=My_FI_Operations/sumd-4  PortSchema="{\"entries\":[{\"content\":{\"sides\":[{\"content\":{\"connectorIds\":[\"In1\"]},\"type\":\"ConnectorPlacement.EquallySpacedRectSide\",\"uuid\":\"423828e0-6700-4575-ac06-a5fb7cb5569f\"},{\"content\":{\"connectorIds\":[\"In2\"],\"side\":\"RIGHT\"},\"type\":\"ConnectorPlacement.EquallySpacedRectSide\",\"uuid\":\"a42db842-eb55-44f2-8f04-0144bc45d908\"},{\"content\":{\"connectorIds\":[\"Out1\"],\"side\":\"TOP\"},\"type\":\"ConnectorPlacement.EquallySpacedRectSide\",\"uuid\":\"eef5137d-31f0-46b4-a53b-5aa31464a7f9\"},{\"content\":{\"connectorIds\":[],\"side\":\"BOTTOM\"},\"type\":\"ConnectorPlacement.EquallySpacedRectSide\",\"uuid\":\"5eff7df8-0604-41b3-8393-dd6fc39cff62\"}]},\"type\":\"ConnectorPlacement.EquallySpacedConnector\",\"uuid\":\"7dd7fe03-b221-4701-a7b2-6552f08320da\"}],\"packageUris\":[\"http://schema.mathworks.com/mf0/Connector/R2020b\"],\"version\":\"1.0\"}"
      mask Display: disp('+')
  sumin_1 : Subsystem  AncestorBlock=My_FI_Operations/sumin_
      settings: LibrarySourceBlock=My_FI_Operations/sumin_  PortSchema="{\"entries\":[{\"content\":{\"sides\":[{\"content\":{\"connectorIds\":[\"In1\"]},\"type\":\"ConnectorPlacement.EquallySpacedRectSide\",\"uuid\":\"423828e0-6700-4575-ac06-a5fb7cb5569f\"},{\"content\":{\"connectorIds\":[\"Out1\"],\"side\":\"RIGHT\"},\"type\":\"ConnectorPlacement.EquallySpacedRectSide\",\"uuid\":\"a42db842-eb55-44f2-8f04-0144bc45d908\"},{\"content\":{\"connectorIds\":[],\"side\":\"TOP\"},\"type\":\"ConnectorPlacement.EquallySpacedRectSide\",\"uuid\":\"eef5137d-31f0-46b4-a53b-5aa31464a7f9\"},{\"content\":{\"connectorIds\":[\"In2\"],\"side\":\"BOTTOM\"},\"type\":\"ConnectorPlacement.EquallySpacedRectSide\",\"uuid\":\"f3760898-0e2b-4385-8757-2cc61988fa54\"}]},\"type\":\"ConnectorPlacement.EquallySpacedConnector\",\"uuid\":\"7dd7fe03-b221-4701-a7b2-6552f08320da\"}],\"packageUris\":[\"http://schema.mathworks.com/mf0/Connector/R2020b\"],\"version\":\"1.0\"}"
      mask Display: disp('+')
  sumin_2 : Subsystem  AncestorBlock=My_FI_Operations/sumin_
      settings: LibrarySourceBlock=My_FI_Operations/sumin_  PortSchema="{\"entries\":[{\"content\":{\"sides\":[{\"content\":{\"connectorIds\":[\"In1\"]},\"type\":\"ConnectorPlacement.EquallySpacedRectSide\",\"uuid\":\"423828e0-6700-4575-ac06-a5fb7cb5569f\"},{\"content\":{\"connectorIds\":[\"Out1\"],\"side\":\"RIGHT\"},\"type\":\"ConnectorPlacement.EquallySpacedRectSide\",\"uuid\":\"a42db842-eb55-44f2-8f04-0144bc45d908\"},{\"content\":{\"connectorIds\":[],\"side\":\"TOP\"},\"type\":\"ConnectorPlacement.EquallySpacedRectSide\",\"uuid\":\"eef5137d-31f0-46b4-a53b-5aa31464a7f9\"},{\"content\":{\"connectorIds\":[\"In2\"],\"side\":\"BOTTOM\"},\"type\":\"ConnectorPlacement.EquallySpacedRectSide\",\"uuid\":\"f3760898-0e2b-4385-8757-2cc61988fa54\"}]},\"type\":\"ConnectorPlacement.EquallySpacedConnector\",\"uuid\":\"7dd7fe03-b221-4701-a7b2-6552f08320da\"}],\"packageUris\":[\"http://schema.mathworks.com/mf0/Connector/R2020b\"],\"version\":\"1.0\"}"
      mask Display: disp('+')
  sumin_3 : Subsystem  AncestorBlock=My_FI_Operations/sumin_
      settings: LibrarySourceBlock=My_FI_Operations/sumin_  PortSchema="{\"entries\":[{\"content\":{\"sides\":[{\"content\":{\"connectorIds\":[\"In1\"]},\"type\":\"ConnectorPlacement.EquallySpacedRectSide\",\"uuid\":\"423828e0-6700-4575-ac06-a5fb7cb5569f\"},{\"content\":{\"connectorIds\":[\"Out1\"],\"side\":\"RIGHT\"},\"type\":\"ConnectorPlacement.EquallySpacedRectSide\",\"uuid\":\"a42db842-eb55-44f2-8f04-0144bc45d908\"},{\"content\":{\"connectorIds\":[],\"side\":\"TOP\"},\"type\":\"ConnectorPlacement.EquallySpacedRectSide\",\"uuid\":\"eef5137d-31f0-46b4-a53b-5aa31464a7f9\"},{\"content\":{\"connectorIds\":[\"In2\"],\"side\":\"BOTTOM\"},\"type\":\"ConnectorPlacement.EquallySpacedRectSide\",\"uuid\":\"f3760898-0e2b-4385-8757-2cc61988fa54\"}]},\"type\":\"ConnectorPlacement.EquallySpacedConnector\",\"uuid\":\"7dd7fe03-b221-4701-a7b2-6552f08320da\"}],\"packageUris\":[\"http://schema.mathworks.com/mf0/Connector/R2020b\"],\"version\":\"1.0\"}"
      mask Display: disp('+')
  sumq-1 : Subsystem  AncestorBlock=My_FI_Operations/sumq-1
      settings: LibrarySourceBlock=My_FI_Operations/sumq-1  PortSchema="{\"entries\":[{\"content\":{\"sides\":[{\"content\":{\"connectorIds\":[]},\"type\":\"ConnectorPlacement.EquallySpacedRectSide\",\"uuid\":\"423828e0-6700-4575-ac06-a5fb7cb5569f\"},{\"content\":{\"connectorIds\":[\"In2\"],\"side\":\"RIGHT\"},\"type\":\"ConnectorPlacement.EquallySpacedRectSide\",\"uuid\":\"a42db842-eb55-44f2-8f04-0144bc45d908\"},{\"content\":{\"connectorIds\":[\"Out1\"],\"side\":\"TOP\"},\"type\":\"ConnectorPlacement.EquallySpacedRectSide\",\"uuid\":\"eef5137d-31f0-46b4-a53b-5aa31464a7f9\"},{\"content\":{\"connectorIds\":[\"In1\"],\"side\":\"BOTTOM\"},\"type\":\"ConnectorPlacement.EquallySpacedRectSide\",\"uuid\":\"2873f229-5340-47da-9b40-109923f96826\"}]},\"type\":\"ConnectorPlacement.EquallySpacedConnector\",\"uuid\":\"7dd7fe03-b221-4701-a7b2-6552f08320da\"}],\"packageUris\":[\"http://schema.mathworks.com/mf0/Connector/R2020b\"],\"version\":\"1.0\"}"
      mask Display: disp('+')
  sumq-2 : Subsystem  AncestorBlock=My_FI_Operations/sumq-2
      settings: LibrarySourceBlock=My_FI_Operations/sumq-2  PortSchema="{\"entries\":[{\"content\":{\"sides\":[{\"content\":{\"connectorIds\":[]},\"type\":\"ConnectorPlacement.EquallySpacedRectSide\",\"uuid\":\"423828e0-6700-4575-ac06-a5fb7cb5569f\"},{\"content\":{\"connectorIds\":[\"In2\"],\"side\":\"RIGHT\"},\"type\":\"ConnectorPlacement.EquallySpacedRectSide\",\"uuid\":\"a42db842-eb55-44f2-8f04-0144bc45d908\"},{\"content\":{\"connectorIds\":[\"Out1\"],\"side\":\"TOP\"},\"type\":\"ConnectorPlacement.EquallySpacedRectSide\",\"uuid\":\"eef5137d-31f0-46b4-a53b-5aa31464a7f9\"},{\"content\":{\"connectorIds\":[\"In1\"],\"side\":\"BOTTOM\"},\"type\":\"ConnectorPlacement.EquallySpacedRectSide\",\"uuid\":\"a9563537-0a55-4c2c-8717-0ee3290f778d\"}]},\"type\":\"ConnectorPlacement.EquallySpacedConnector\",\"uuid\":\"7dd7fe03-b221-4701-a7b2-6552f08320da\"}],\"packageUris\":[\"http://schema.mathworks.com/mf0/Connector/R2020b\"],\"version\":\"1.0\"}"
      mask Display: disp('+')
  sumq-3 : Subsystem  AncestorBlock=My_FI_Operations/sumq-3
      settings: LibrarySourceBlock=My_FI_Operations/sumq-3  PortSchema="{\"entries\":[{\"content\":{\"sides\":[{\"content\":{\"connectorIds\":[\"In1\"]},\"type\":\"ConnectorPlacement.EquallySpacedRectSide\",\"uuid\":\"423828e0-6700-4575-ac06-a5fb7cb5569f\"},{\"content\":{\"connectorIds\":[],\"side\":\"RIGHT\"},\"type\":\"ConnectorPlacement.EquallySpacedRectSide\",\"uuid\":\"a42db842-eb55-44f2-8f04-0144bc45d908\"},{\"content\":{\"connectorIds\":[\"Out1\"],\"side\":\"TOP\"},\"type\":\"ConnectorPlacement.EquallySpacedRectSide\",\"uuid\":\"eef5137d-31f0-46b4-a53b-5aa31464a7f9\"},{\"content\":{\"connectorIds\":[\"In2\"],\"side\":\"BOTTOM\"},\"type\":\"ConnectorPlacement.EquallySpacedRectSide\",\"uuid\":\"7a6dc86a-9d1e-447c-8c0e-423c8e5484b3\"}]},\"type\":\"ConnectorPlacement.EquallySpacedConnector\",\"uuid\":\"7dd7fe03-b221-4701-a7b2-6552f08320da\"}],\"packageUris\":[\"http://schema.mathworks.com/mf0/Connector/R2020b\"],\"version\":\"1.0\"}"
      mask Display: disp('+')
  Out1 : Outport
  wires:
  Delay77/1 -> sumin_1/1(In1)
  Delay42/1 -> multb6_1/2(In1), Delay43/1
  multb6_2/1(Out1) -> sumb6_2/2(In1)
  Delay53/1 -> Rate Transition1/1, Rate Transition3/1, Delay57/1, Delay55/1
  Delay78/1 -> sumin_2/1(In1)
  sumin_2/1(Out1) -> multa2_2/2(In1), multa4_2/2(In1), multa6_2/2(In1), multa8_2/2(In1), multa10_2/2(In1), multa12_2/2(In1), Zero-Order Hold7/1
  b0_6/1 -> multb12_3/1(In2)
  Delay69/1 -> Delay70/1
  Delay101/1 -> sumd-4/1(In1)
  Delay31/1 -> multb0_1/2(In1), Delay41/1
  sumq-2/1(Out1) -> sumin_2/2(In2)
  Delay32/1 -> multb6_2/2(In1), Delay33/1
  multa8_3/1(Out1) -> Delay88/1
  multb6_1/1(Out1) -> sumb6_1/2(In1)
  Delay94/1 -> suma2_1/2(In1)
  Delay68/1 -> multb4_3/2(In1), Delay69/1
  Delay41/1 -> Delay42/1
  Delay85/1 -> Delay81/1
  Zero-Order Hold/1 -> Delay77/1
  Delay64/1 -> Delay65/1
  b2_4/1 -> multb10_2/1(In2)
  sumin_1/1(Out1) -> multa2_1/2(In1), multa4_1/2(In1), multa6_1/2(In1), multa8_1/2(In1), multa10_1/2(In1), multa12_1/2(In1), Zero-Order Hold6/1
  sumb4_3/1(Out1) -> sumb6_3/1(In2)
  b4_5/1 -> multb4_3/1(In2)
  Zero-Order Hold2/1 -> Delay109/1
  Zero-Order Hold1/1 -> Delay78/1
  Delay84/1 -> suma2_3/2(In1)
  Delay27/1 -> multb0_2/2(In1), Delay30/1
  in/1 -> Delay53/1, Rate Transition/1
  Delay100/1 -> Delay97/1
  multa2_3/1(Out1) -> suma2_3/1(In2)
  Delay65/1 -> multb6_3/2(In1), Delay66/1
  Delay28/1 -> Delay35/1
  Delay33/1 -> Delay34/1
  Delay57/1 -> Rate Transition4/1, Rate Transition6/1, Delay74/1, Delay59/1
  Delay48/1 -> Delay52/1
  Delay98/1 -> Delay94/1
  multa10_2/1(Out1) -> Delay75/1
  Delay40/1 -> multb2_1/2(In1), Delay49/1
  Delay13/1 -> Delay23/1
  a10_2/1 -> multa10_2/1(In2)
  sumb2_3/1(Out1) -> sumb4_3/1(In2)
  a4_3/1 -> multa4_3/1(In2)
  sumd-3/1(Out1) -> sumq-2/1(In1)
  suma6_3/1(Out1) -> Delay85/1
  sumb12_1/1(Out1) -> Zero-Order Hold/1
  Delay63/1 -> multb2_3/2(In1), Delay71/1
  Multiport Switch1/1 -> Out1/1
  a12_1/1 -> multa12_1/1(In2)
  multb4_3/1(Out1) -> sumb4_3/2(In1)
  multa8_2/1(Out1) -> Delay15/1
  sumq-3/1(Out1) -> sumin_3/2(In2)
  Constant82/1 -> Sum4/2
  Delay15/1 -> Delay104/1
  Delay109/1 -> sumin_3/1(In1)
  Delay86/1 -> sumq-3/1(In1)
  multa4_2/1(Out1) -> suma4_2/1(In1)
  sumd-4/1(Out1) -> sumq-3/2(In2)
  b0_1/1 -> multb0_1/1(In2)
  Delay88/1 -> Delay84/1
  multa6_3/1(Out1) -> suma6_3/1(In1)
  Counter Limited1/1 -> Sum4/1
  sumb6_2/1(Out1) -> sumb8_2/1(In2)
  sumb8_3/1(Out1) -> sumb10_3/1(In2)
  Delay61/1 -> multb0_3/2(In1), Delay64/1
  Delay91/1 -> sumd-2/2(In2)
  multa4_3/1(Out1) -> suma4_3/1(In1)
  a2_3/1 -> multa2_3/1(In2)
  a10_3/1 -> multa10_3/1(In2)
  a12_3/1 -> multa12_3/1(In2)
  b0_2/1 -> multb12_1/1(In2)
  a12_2/1 -> multa12_2/1(In2)
  Delay95/1 -> Delay91/1
  multb12_1/1(Out1) -> sumb12_1/2(In1)
  b2_2/1 -> multb10_1/1(In2)
  a6_3/1 -> multa6_3/1(In2)
  sumin_3/1(Out1) -> multa2_3/2(In1), multa4_3/2(In1), multa6_3/2(In1), multa8_3/2(In1), multa10_3/2(In1), multa12_3/2(In1), Zero-Order Hold8/1
  Delay62/1 -> Delay68/1
  Delay70/1 -> multb10_3/2(In1)
  a4_1/1 -> multa4_1/1(In2)
  Delay74/1 -> Rate Transition7/1, Delay76/1
  Delay50/1 -> multb8_1/2(In1)
  sumd-2/1(Out1) -> sumq-1/1(In2)
  a2_1/1 -> multa2_1/1(In2)
  sumb8_1/1(Out1) -> sumb10_1/1(In2)
  Delay14/1 -> suma4_2/2(In2)
  Delay87/1 -> suma4_3/2(In2)
  a4_2/1 -> multa4_2/1(In2)
  Zero-Order Hold6/1 -> Rate Transition12/1
  Subtract2/1 -> Multiport Switch1/1
  a6_2/1 -> multa6_2/1(In2)
  multb2_3/1(Out1) -> sumb2_3/2(In1)
  multb4_1/1(Out1) -> sumb4_1/2(In1)
  Delay81/1 -> sumd-4/2(In2)
  Delay89/1 -> suma6_3/2(In2)
  Delay35/1 -> multb4_2/2(In1), Delay36/1
  Delay34/1 -> multb12_2/2(In1)
  multb2_1/1(Out1) -> sumb2_1/2(In1)
  multb6_3/1(Out1) -> sumb6_3/2(In1)
  a8_1/1 -> multa8_1/1(In2)
  Delay52/1 -> multb8_2/2(In1)
  sumq-1/1(Out1) -> sumin_1/2(In2)
  b6_3/1 -> multb6_3/1(In2)
  sumb10_3/1(Out1) -> sumb12_3/1(In2)
  multb8_3/1(Out1) -> sumb8_3/2(In1)
  a2_2/1 -> multa2_2/1(In2)
  Delay55/1 -> Rate Transition2/1
  Delay93/1 -> Delay86/1
  multa10_3/1(Out1) -> Delay90/1
  multb10_3/1(Out1) -> sumb10_3/2(In1)
  Delay60/1 -> suma6_2/2(In2)
  suma2_3/1(Out1) -> sumd-2/1(In1)
  Delay30/1 -> Delay32/1
  sumb4_1/1(Out1) -> sumb6_1/1(In2)
  multb2_2/1(Out1) -> sumb2_2/2(In1)
  b2_1/1 -> multb2_1/1(In2)
  Delay23/1 -> sumd-3/2(In2)
  b4_1/1 -> multb4_1/1(In2)
  multb10_1/1(Out1) -> sumb10_1/2(In1)
  Delay47/1 -> multb10_1/2(In1)
  Delay103/1 -> sumq-1/2(In1)
  Constant102/1 -> Subtract2/1
  Delay36/1 -> Delay37/1
  sumb10_1/1(Out1) -> sumb12_1/1(In2)
  b6_2/1 -> multb6_2/1(In2)
  b6_1/1 -> multb6_1/1(In2)
  b0_4/1 -> multb12_2/1(In2)
  multb8_1/1(Out1) -> sumb8_1/2(In1)
  Delay29/1 -> multb2_2/2(In1), Delay48/1
  b4_2/1 -> multb8_1/1(In2)
  Delay59/1 -> Rate Transition5/1
  b2_6/1 -> multb10_3/1(In2)
  sumb2_2/1(Out1) -> sumb4_2/1(In2)
  multb4_2/1(Out1) -> sumb4_2/2(In1)
  Delay71/1 -> Delay72/1
  multb0_2/1(Out1) -> sumb2_2/1(In2)
  sumb4_2/1(Out1) -> sumb6_2/1(In2)
  multb8_2/1(Out1) -> sumb8_2/2(In1)
  multb12_2/1(Out1) -> sumb12_2/2(In1)
  sumb8_2/1(Out1) -> sumb10_2/1(In2)
  multb10_2/1(Out1) -> sumb10_2/2(In1)
  b0_3/1 -> multb0_2/1(In2)
  suma2_1/1(Out1) -> Delay102/1
  b2_3/1 -> multb2_2/1(In2)
  Delay39/1 -> Delay45/1
  b4_6/1 -> multb8_3/1(In2)
  Delay66/1 -> Delay67/1
  multb12_3/1(Out1) -> sumb12_3/2(In1)
  sumb6_3/1(Out1) -> sumb8_3/1(In2)
  Delay67/1 -> multb12_3/2(In1)
  suma2_2/1(Out1) -> Delay101/1
  suma4_3/1(Out1) -> Delay82/1
  multa6_2/1(Out1) -> suma6_2/1(In1)
  suma4_2/1(Out1) -> Delay103/1
  Delay104/1 -> suma2_2/2(In1)
  Delay99/1 -> suma6_1/2(In2)
  Delay80/1 -> Delay89/1
  sumb2_1/1(Out1) -> sumb4_1/1(In2)
  multa12_1/1(Out1) -> Delay105/1
  a10_1/1 -> multa10_1/1(In2)
  multa10_1/1(Out1) -> Delay100/1
  Delay44/1 -> multb12_1/2(In1)
  Delay82/1 -> sumq-2/2(In2)
  multa12_3/1(Out1) -> Delay80/1
  Delay90/1 -> Delay87/1
  Delay75/1 -> Delay14/1
  Zero-Order Hold7/1 -> Rate Transition9/1
  suma6_1/1(Out1) -> Delay95/1
  Zero-Order Hold8/1 -> Rate Transition10/1
  sumb10_2/1(Out1) -> sumb12_2/1(In2)
  sumb12_2/1(Out1) -> Zero-Order Hold1/1
  multb0_3/1(Out1) -> sumb2_3/1(In2)
  multa12_2/1(Out1) -> Delay92/1
  Delay105/1 -> Delay99/1
  Delay45/1 -> multb4_1/2(In1), Delay46/1
  multa2_1/1(Out1) -> suma2_1/1(In2)
  multa4_1/1(Out1) -> suma4_1/1(In1)
  Delay102/1 -> sumd-3/1(In1)
  Delay92/1 -> Delay60/1
  a8_2/1 -> multa8_2/1(In2)
  b0_5/1 -> multb0_3/1(In2)
  Delay72/1 -> multb8_3/2(In1)
  Delay97/1 -> suma4_1/2(In2)
  b4_4/1 -> multb8_2/1(In2)
  multa6_1/1(Out1) -> suma6_1/1(In1)
  sumb12_3/1(Out1) -> Zero-Order Hold2/1
  suma6_2/1(Out1) -> Delay13/1
  a6_1/1 -> multa6_1/1(In2)
  Delay37/1 -> multb10_2/2(In1)
  Delay43/1 -> Delay44/1
  multa2_2/1(Out1) -> suma2_2/1(In2)
  Sum4/1 -> Subtract2/2
  multa8_1/1(Out1) -> Delay98/1
  Delay76/1 -> Rate Transition8/1
  suma4_1/1(Out1) -> Delay93/1
  multb0_1/1(Out1) -> sumb2_1/1(In2)
  b4_3/1 -> multb4_2/1(In2)
  b2_5/1 -> multb2_3/1(In2)
  a8_3/1 -> multa8_3/1(In2)
  Delay46/1 -> Delay47/1
  sumb6_1/1(Out1) -> sumb8_1/1(In2)
  Delay49/1 -> Delay50/1
  Rate Transition/1 -> Delay31/1
  Rate Transition1/1 -> Delay39/1
  Rate Transition2/1 -> Delay40/1
  Rate Transition3/1 -> Delay27/1
  Rate Transition4/1 -> Delay28/1
  Rate Transition5/1 -> Delay29/1
  Rate Transition6/1 -> Delay61/1
  Rate Transition7/1 -> Delay62/1
  Rate Transition8/1 -> Delay63/1
  Rate Transition12/1 -> Multiport Switch1/2
  Rate Transition9/1 -> Multiport Switch1/3
  Rate Transition10/1 -> Multiport Switch1/4
